simulink model "FullCarLateral"  (R2023b)
settings: Solver=FixedStepAuto  StartTime=0.0  StopTime=30  FixedStep=dt  MaxStep=0.001  RelTol=1e-3
model workspace (MAT data in the model file):
  AMU = Simulink.Signal
  AMU.DataType = 'double'
  AMU.Dimensions = 1
  AMU.DimensionsMode = 'auto'
  AMU.Complexity = 'real'
  AMU.SampleTime = -1
  AMU.SamplingMode = 'auto'
  EPSILON = Simulink.Signal
  EPSILON.DataType = 'double'
  EPSILON.Dimensions = 1
  EPSILON.DimensionsMode = 'auto'
  EPSILON.Complexity = 'real'
  EPSILON.SampleTime = -1
  EPSILON.SamplingMode = 'auto'
  FZO = Simulink.Signal
  FZO.DataType = 'double'
  FZO.Dimensions = 1
  FZO.DimensionsMode = 'auto'
  FZO.Complexity = 'real'
  FZO.SampleTime = -1
  FZO.SamplingMode = 'auto'
  LCX = Simulink.Signal
  LCX.DataType = 'double'
  LCX.Dimensions = 1
  LCX.DimensionsMode = 'auto'
  LCX.Complexity = 'real'
  LCX.SampleTime = -1
  LCX.SamplingMode = 'auto'
  LCY = Simulink.Signal
  LCY.DataType = 'double'
  LCY.Dimensions = 1
  LCY.DimensionsMode = 'auto'
  LCY.Complexity = 'real'
  LCY.SampleTime = -1
  LCY.SamplingMode = 'auto'
  LCZ = Simulink.Signal
  LCZ.DataType = 'double'
  LCZ.Dimensions = 1
  LCZ.DimensionsMode = 'auto'
  LCZ.Complexity = 'real'
  LCZ.SampleTime = -1
  LCZ.SamplingMode = 'auto'
  LEX = Simulink.Signal
  LEX.DataType = 'double'
  LEX.Dimensions = 1
  LEX.DimensionsMode = 'auto'
  LEX.Complexity = 'real'
  LEX.SampleTime = -1
  LEX.SamplingMode = 'auto'
  LEY = Simulink.Signal
  LEY.DataType = 'double'
  LEY.Dimensions = 1
  LEY.DimensionsMode = 'auto'
  LEY.Complexity = 'real'
  LEY.SampleTime = -1
  LEY.SamplingMode = 'auto'
  LFZO = Simulink.Signal
  LFZO.DataType = 'double'
  LFZO.Dimensions = 1
  LFZO.DimensionsMode = 'auto'
  LFZO.Complexity = 'real'
  LFZO.SampleTime = -1
  LFZO.SamplingMode = 'auto'
  LHX = Simulink.Signal
  LHX.DataType = 'double'
  LHX.Dimensions = 1
  LHX.DimensionsMode = 'auto'
  LHX.Complexity = 'real'
  LHX.SampleTime = -1
  LHX.SamplingMode = 'auto'
  LHY = Simulink.Signal
  LHY.DataType = 'double'
  LHY.Dimensions = 1
  LHY.DimensionsMode = 'auto'
  LHY.Complexity = 'real'
  LHY.SampleTime = -1
  LHY.SamplingMode = 'auto'
  LKXKAPPA = Simulink.Signal
  LKXKAPPA.DataType = 'double'
  LKXKAPPA.Dimensions = 1
  LKXKAPPA.DimensionsMode = 'auto'
  LKXKAPPA.Complexity = 'real'
  LKXKAPPA.SampleTime = -1
  LKXKAPPA.SamplingMode = 'auto'
  LKYALPHA = Simulink.Signal
  LKYALPHA.DataType = 'double'
  LKYALPHA.Dimensions = 1
  LKYALPHA.DimensionsMode = 'auto'
  LKYALPHA.Complexity = 'real'
  LKYALPHA.SampleTime = -1
  LKYALPHA.SamplingMode = 'auto'
  LKYGAMMA = Simulink.Signal
  LKYGAMMA.DataType = 'double'
  LKYGAMMA.Dimensions = 1
  LKYGAMMA.DimensionsMode = 'auto'
  LKYGAMMA.Complexity = 'real'
  LKYGAMMA.SampleTime = -1
  LKYGAMMA.SamplingMode = 'auto'
  LKZGAMMA = Simulink.Signal
  LKZGAMMA.DataType = 'double'
  LKZGAMMA.Dimensions = 1
  LKZGAMMA.DimensionsMode = 'auto'
  LKZGAMMA.Complexity = 'real'
  LKZGAMMA.SampleTime = -1
  LKZGAMMA.SamplingMode = 'auto'
  LMR = Simulink.Signal
  LMR.DataType = 'double'
  LMR.Dimensions = 1
  LMR.DimensionsMode = 'auto'
  LMR.Complexity = 'real'
  LMR.SampleTime = -1
  LMR.SamplingMode = 'auto'
  LMUV = Simulink.Signal
  LMUV.DataType = 'double'
  LMUV.Dimensions = 1
  LMUV.DimensionsMode = 'auto'
  LMUV.Complexity = 'real'
  LMUV.SampleTime = -1
  LMUV.SamplingMode = 'auto'
  LMUX = Simulink.Signal
  LMUX.DataType = 'double'
  LMUX.Dimensions = 1
  LMUX.DimensionsMode = 'auto'
  LMUX.Complexity = 'real'
  LMUX.SampleTime = -1
  LMUX.SamplingMode = 'auto'
  LMUXAST = Simulink.Signal
  LMUXAST.DataType = 'double'
  LMUXAST.Dimensions = 1
  LMUXAST.DimensionsMode = 'auto'
  LMUXAST.Complexity = 'real'
  LMUXAST.SampleTime = -1
  LMUXAST.SamplingMode = 'auto'
  LMUXPRIME = Simulink.Signal
  LMUXPRIME.DataType = 'double'
  LMUXPRIME.Dimensions = 1
  LMUXPRIME.DimensionsMode = 'auto'
  LMUXPRIME.Complexity = 'real'
  LMUXPRIME.SampleTime = -1
  LMUXPRIME.SamplingMode = 'auto'
  LMUY = Simulink.Signal
  LMUY.DataType = 'double'
  LMUY.Dimensions = 1
  LMUY.DimensionsMode = 'auto'
  LMUY.Complexity = 'real'
  LMUY.SampleTime = -1
  LMUY.SamplingMode = 'auto'
  LMUYAST = Simulink.Signal
  LMUYAST.DataType = 'double'
  LMUYAST.Dimensions = 1
  LMUYAST.DimensionsMode = 'auto'
  LMUYAST.Complexity = 'real'
  LMUYAST.SampleTime = -1
  LMUYAST.SamplingMode = 'auto'
  LMUYPRIME = Simulink.Signal
  LMUYPRIME.DataType = 'double'
  LMUYPRIME.Dimensions = 1
  LMUYPRIME.DimensionsMode = 'auto'
  LMUYPRIME.Complexity = 'real'
  LMUYPRIME.SampleTime = -1
  LMUYPRIME.SamplingMode = 'auto'
  LMX = Simulink.Signal
  LMX.DataType = 'double'
  LMX.Dimensions = 1
  LMX.DimensionsMode = 'auto'
  LMX.Complexity = 'real'
  LMX.SampleTime = -1
  LMX.SamplingMode = 'auto'
  LMY = Simulink.Signal
  LMY.DataType = 'double'
  LMY.Dimensions = 1
  LMY.DimensionsMode = 'auto'
  LMY.Complexity = 'real'
  LMY.SampleTime = -1
  LMY.SamplingMode = 'auto'
  LS = Simulink.Signal
  LS.DataType = 'double'
  LS.Dimensions = 1
  LS.DimensionsMode = 'auto'
  LS.Complexity = 'real'
  LS.SampleTime = -1
  LS.SamplingMode = 'auto'
  LT = Simulink.Signal
  LT.DataType = 'double'
  LT.Dimensions = 1
  LT.DimensionsMode = 'auto'
  LT.Complexity = 'real'
  LT.SampleTime = -1
  LT.SamplingMode = 'auto'
  LVX = Simulink.Signal
  LVX.DataType = 'double'
  LVX.Dimensions = 1
  LVX.DimensionsMode = 'auto'
  LVX.Complexity = 'real'
  LVX.SampleTime = -1
  LVX.SamplingMode = 'auto'
  LVY = Simulink.Signal
  LVY.DataType = 'double'
  LVY.Dimensions = 1
  LVY.DimensionsMode = 'auto'
  LVY.Complexity = 'real'
  LVY.SampleTime = -1
  LVY.SamplingMode = 'auto'
  LVYKAPPA = Simulink.Signal
  LVYKAPPA.DataType = 'double'
  LVYKAPPA.Dimensions = 1
  LVYKAPPA.DimensionsMode = 'auto'
  LVYKAPPA.Complexity = 'real'
  LVYKAPPA.SampleTime = -1
  LVYKAPPA.SamplingMode = 'auto'
  LXALPHA = Simulink.Signal
  LXALPHA.DataType = 'double'
  LXALPHA.Dimensions = 1
  LXALPHA.DimensionsMode = 'auto'
  LXALPHA.Complexity = 'real'
  LXALPHA.SampleTime = -1
  LXALPHA.SamplingMode = 'auto'
  LYKAPPA = Simulink.Signal
  LYKAPPA.DataType = 'double'
  LYKAPPA.Dimensions = 1
  LYKAPPA.DimensionsMode = 'auto'
  LYKAPPA.Complexity = 'real'
  LYKAPPA.SampleTime = -1
  LYKAPPA.SamplingMode = 'auto'
  PCX1 = Simulink.Signal
  PCX1.DataType = 'double'
  PCX1.Dimensions = 1
  PCX1.DimensionsMode = 'auto'
  PCX1.Complexity = 'real'
  PCX1.SampleTime = -1
  PCX1.SamplingMode = 'auto'
  PCY1 = Simulink.Signal
  PCY1.DataType = 'double'
  PCY1.Dimensions = 1
  PCY1.DimensionsMode = 'auto'
  PCY1.Complexity = 'real'
  PCY1.SampleTime = -1
  PCY1.SamplingMode = 'auto'
  PDX1 = Simulink.Signal
  PDX1.DataType = 'double'
  PDX1.Dimensions = 1
  PDX1.DimensionsMode = 'auto'
  PDX1.Complexity = 'real'
  PDX1.SampleTime = -1
  PDX1.SamplingMode = 'auto'
  PDX2 = Simulink.Signal
  PDX2.DataType = 'double'
  PDX2.Dimensions = 1
  PDX2.DimensionsMode = 'auto'
  PDX2.Complexity = 'real'
  PDX2.SampleTime = -1
  PDX2.SamplingMode = 'auto'
  PDX3 = Simulink.Signal
  PDX3.DataType = 'double'
  PDX3.Dimensions = 1
  PDX3.DimensionsMode = 'auto'
  PDX3.Complexity = 'real'
  PDX3.SampleTime = -1
  PDX3.SamplingMode = 'auto'
  PDY1 = Simulink.Signal
  PDY1.DataType = 'double'
  PDY1.Dimensions = 1
  PDY1.DimensionsMode = 'auto'
  PDY1.Complexity = 'real'
  PDY1.SampleTime = -1
  PDY1.SamplingMode = 'auto'
  PDY2 = Simulink.Signal
  PDY2.DataType = 'double'
  PDY2.Dimensions = 1
  PDY2.DimensionsMode = 'auto'
  PDY2.Complexity = 'real'
  PDY2.SampleTime = -1
  PDY2.SamplingMode = 'auto'
  PDY3 = Simulink.Signal
  PDY3.DataType = 'double'
  PDY3.Dimensions = 1
  PDY3.DimensionsMode = 'auto'
  PDY3.Complexity = 'real'
  PDY3.SampleTime = -1
  PDY3.SamplingMode = 'auto'
  PEX1 = Simulink.Signal
  PEX1.DataType = 'double'
  PEX1.Dimensions = 1
  PEX1.DimensionsMode = 'auto'
  PEX1.Complexity = 'real'
  PEX1.SampleTime = -1
  PEX1.SamplingMode = 'auto'
  PEX2 = Simulink.Signal
  PEX2.DataType = 'double'
  PEX2.Dimensions = 1
  PEX2.DimensionsMode = 'auto'
  PEX2.Complexity = 'real'
  PEX2.SampleTime = -1
  PEX2.SamplingMode = 'auto'
  PEX3 = Simulink.Signal
  PEX3.DataType = 'double'
  PEX3.Dimensions = 1
  PEX3.DimensionsMode = 'auto'
  PEX3.Complexity = 'real'
  PEX3.SampleTime = -1
  PEX3.SamplingMode = 'auto'
  PEX4 = Simulink.Signal
  PEX4.DataType = 'double'
  PEX4.Dimensions = 1
  PEX4.DimensionsMode = 'auto'
  PEX4.Complexity = 'real'
  PEX4.SampleTime = -1
  PEX4.SamplingMode = 'auto'
  PEY1 = Simulink.Signal
  PEY1.DataType = 'double'
  PEY1.Dimensions = 1
  PEY1.DimensionsMode = 'auto'
  PEY1.Complexity = 'real'
  PEY1.SampleTime = -1
  PEY1.SamplingMode = 'auto'
  PEY2 = Simulink.Signal
  PEY2.DataType = 'double'
  PEY2.Dimensions = 1
  PEY2.DimensionsMode = 'auto'
  PEY2.Complexity = 'real'
  PEY2.SampleTime = -1
  PEY2.SamplingMode = 'auto'
  PEY3 = Simulink.Signal
  PEY3.DataType = 'double'
  PEY3.Dimensions = 1
  PEY3.DimensionsMode = 'auto'
  PEY3.Complexity = 'real'
  PEY3.SampleTime = -1
  PEY3.SamplingMode = 'auto'
  PEY4 = Simulink.Signal
  PEY4.DataType = 'double'
  PEY4.Dimensions = 1
  PEY4.DimensionsMode = 'auto'
  PEY4.Complexity = 'real'
  PEY4.SampleTime = -1
  PEY4.SamplingMode = 'auto'
  PEY5 = Simulink.Signal
  PEY5.DataType = 'double'
  PEY5.Dimensions = 1
  PEY5.DimensionsMode = 'auto'
  PEY5.Complexity = 'real'
  PEY5.SampleTime = -1
  PEY5.SamplingMode = 'auto'
  PHX1 = Simulink.Signal
  PHX1.DataType = 'double'
  PHX1.Dimensions = 1
  PHX1.DimensionsMode = 'auto'
  PHX1.Complexity = 'real'
  PHX1.SampleTime = -1
  PHX1.SamplingMode = 'auto'
  PHX2 = Simulink.Signal
  PHX2.DataType = 'double'
  PHX2.Dimensions = 1
  PHX2.DimensionsMode = 'auto'
  PHX2.Complexity = 'real'
  PHX2.SampleTime = -1
  PHX2.SamplingMode = 'auto'
  PHY1 = Simulink.Signal
  PHY1.DataType = 'double'
  PHY1.Dimensions = 1
  PHY1.DimensionsMode = 'auto'
  PHY1.Complexity = 'real'
  PHY1.SampleTime = -1
  PHY1.SamplingMode = 'auto'
  PHY2 = Simulink.Signal
  PHY2.DataType = 'double'
  PHY2.Dimensions = 1
  PHY2.DimensionsMode = 'auto'
  PHY2.Complexity = 'real'
  PHY2.SampleTime = -1
  PHY2.SamplingMode = 'auto'
  PKX1 = Simulink.Signal
  PKX1.DataType = 'double'
  PKX1.Dimensions = 1
  PKX1.DimensionsMode = 'auto'
  PKX1.Complexity = 'real'
  PKX1.SampleTime = -1
  PKX1.SamplingMode = 'auto'
  PKX2 = Simulink.Signal
  PKX2.DataType = 'double'
  PKX2.Dimensions = 1
  PKX2.DimensionsMode = 'auto'
  PKX2.Complexity = 'real'
  PKX2.SampleTime = -1
  PKX2.SamplingMode = 'auto'
  PKX3 = Simulink.Signal
  PKX3.DataType = 'double'
  PKX3.Dimensions = 1
  PKX3.DimensionsMode = 'auto'
  PKX3.Complexity = 'real'
  PKX3.SampleTime = -1
  PKX3.SamplingMode = 'auto'
  PKY1 = Simulink.Signal
  PKY1.DataType = 'double'
  PKY1.Dimensions = 1
  PKY1.DimensionsMode = 'auto'
  PKY1.Complexity = 'real'
  PKY1.SampleTime = -1
  PKY1.SamplingMode = 'auto'
  PKY2 = Simulink.Signal
  PKY2.DataType = 'double'
  PKY2.Dimensions = 1
  PKY2.DimensionsMode = 'auto'
  PKY2.Complexity = 'real'
  PKY2.SampleTime = -1
  PKY2.SamplingMode = 'auto'
  PKY3 = Simulink.Signal
  PKY3.DataType = 'double'
  PKY3.Dimensions = 1
  PKY3.DimensionsMode = 'auto'
  PKY3.Complexity = 'real'
  PKY3.SampleTime = -1
  PKY3.SamplingMode = 'auto'
  PKY4 = Simulink.Signal
  PKY4.DataType = 'double'
  PKY4.Dimensions = 1
  PKY4.DimensionsMode = 'auto'
  PKY4.Complexity = 'real'
  PKY4.SampleTime = -1
  PKY4.SamplingMode = 'auto'
  PKY5 = Simulink.Signal
  PKY5.DataType = 'double'
  PKY5.Dimensions = 1
  PKY5.DimensionsMode = 'auto'
  PKY5.Complexity = 'real'
  PKY5.SampleTime = -1
  PKY5.SamplingMode = 'auto'
  PKY6 = Simulink.Signal
  PKY6.DataType = 'double'
  PKY6.Dimensions = 1
  PKY6.DimensionsMode = 'auto'
  PKY6.Complexity = 'real'
  PKY6.SampleTime = -1
  PKY6.SamplingMode = 'auto'
  PKY7 = Simulink.Signal
  PKY7.DataType = 'double'
  PKY7.Dimensions = 1
  PKY7.DimensionsMode = 'auto'
  PKY7.Complexity = 'real'
  PKY7.SampleTime = -1
  PKY7.SamplingMode = 'auto'
  PVX1 = Simulink.Signal
  PVX1.DataType = 'double'
  PVX1.Dimensions = 1
  PVX1.DimensionsMode = 'auto'
  PVX1.Complexity = 'real'
  PVX1.SampleTime = -1
  PVX1.SamplingMode = 'auto'
  PVX2 = Simulink.Signal
  PVX2.DataType = 'double'
  PVX2.Dimensions = 1
  PVX2.DimensionsMode = 'auto'
  PVX2.Complexity = 'real'
  PVX2.SampleTime = -1
  PVX2.SamplingMode = 'auto'
  PVY1 = Simulink.Signal
  PVY1.DataType = 'double'
  PVY1.Dimensions = 1
  PVY1.DimensionsMode = 'auto'
  PVY1.Complexity = 'real'
  PVY1.SampleTime = -1
  PVY1.SamplingMode = 'auto'
  PVY2 = Simulink.Signal
  PVY2.DataType = 'double'
  PVY2.Dimensions = 1
  PVY2.DimensionsMode = 'auto'
  PVY2.Complexity = 'real'
  PVY2.SampleTime = -1
  PVY2.SamplingMode = 'auto'
  PVY3 = Simulink.Signal
  PVY3.DataType = 'double'
  PVY3.Dimensions = 1
  PVY3.DimensionsMode = 'auto'
  PVY3.Complexity = 'real'
  PVY3.SampleTime = -1
  PVY3.SamplingMode = 'auto'
  PVY4 = Simulink.Signal
  PVY4.DataType = 'double'
  PVY4.Dimensions = 1
  PVY4.DimensionsMode = 'auto'
  PVY4.Complexity = 'real'
  PVY4.SampleTime = -1
  PVY4.SamplingMode = 'auto'
  QBZ1 = Simulink.Signal
  QBZ1.DataType = 'double'
  QBZ1.Dimensions = 1
  QBZ1.DimensionsMode = 'auto'
  QBZ1.Complexity = 'real'
  QBZ1.SampleTime = -1
  QBZ1.SamplingMode = 'auto'
  QBZ10 = Simulink.Signal
  QBZ10.DataType = 'double'
  QBZ10.Dimensions = 1
  QBZ10.DimensionsMode = 'auto'
  QBZ10.Complexity = 'real'
  QBZ10.SampleTime = -1
  QBZ10.SamplingMode = 'auto'
  QBZ2 = Simulink.Signal
  QBZ2.DataType = 'double'
  QBZ2.Dimensions = 1
  QBZ2.DimensionsMode = 'auto'
  QBZ2.Complexity = 'real'
  QBZ2.SampleTime = -1
  QBZ2.SamplingMode = 'auto'
  QBZ3 = Simulink.Signal
  QBZ3.DataType = 'double'
  QBZ3.Dimensions = 1
  QBZ3.DimensionsMode = 'auto'
  QBZ3.Complexity = 'real'
  QBZ3.SampleTime = -1
  QBZ3.SamplingMode = 'auto'
  QBZ5 = Simulink.Signal
  QBZ5.DataType = 'double'
  QBZ5.Dimensions = 1
  QBZ5.DimensionsMode = 'auto'
  QBZ5.Complexity = 'real'
  QBZ5.SampleTime = -1
  QBZ5.SamplingMode = 'auto'
  QBZ6 = Simulink.Signal
  QBZ6.DataType = 'double'
  QBZ6.Dimensions = 1
  QBZ6.DimensionsMode = 'auto'
  QBZ6.Complexity = 'real'
  QBZ6.SampleTime = -1
  QBZ6.SamplingMode = 'auto'
  QBZ9 = Simulink.Signal
  QBZ9.DataType = 'double'
  QBZ9.Dimensions = 1
  QBZ9.DimensionsMode = 'auto'
  QBZ9.Complexity = 'real'
  QBZ9.SampleTime = -1
  QBZ9.SamplingMode = 'auto'
  QCZ1 = Simulink.Signal
  QCZ1.DataType = 'double'
  QCZ1.Dimensions = 1
  QCZ1.DimensionsMode = 'auto'
  QCZ1.Complexity = 'real'
  QCZ1.SampleTime = -1
  QCZ1.SamplingMode = 'auto'
  QDZ1 = Simulink.Signal
  QDZ1.DataType = 'double'
  QDZ1.Dimensions = 1
  QDZ1.DimensionsMode = 'auto'
  QDZ1.Complexity = 'real'
  QDZ1.SampleTime = -1
  QDZ1.SamplingMode = 'auto'
  QDZ10 = Simulink.Signal
  QDZ10.DataType = 'double'
  QDZ10.Dimensions = 1
  QDZ10.DimensionsMode = 'auto'
  QDZ10.Complexity = 'real'
  QDZ10.SampleTime = -1
  QDZ10.SamplingMode = 'auto'
  QDZ11 = Simulink.Signal
  QDZ11.DataType = 'double'
  QDZ11.Dimensions = 1
  QDZ11.DimensionsMode = 'auto'
  QDZ11.Complexity = 'real'
  QDZ11.SampleTime = -1
  QDZ11.SamplingMode = 'auto'
  QDZ2 = Simulink.Signal
  QDZ2.DataType = 'double'
  QDZ2.Dimensions = 1
  QDZ2.DimensionsMode = 'auto'
  QDZ2.Complexity = 'real'
  QDZ2.SampleTime = -1
  QDZ2.SamplingMode = 'auto'
  QDZ3 = Simulink.Signal
  QDZ3.DataType = 'double'
  QDZ3.Dimensions = 1
  QDZ3.DimensionsMode = 'auto'
  QDZ3.Complexity = 'real'
  QDZ3.SampleTime = -1
  QDZ3.SamplingMode = 'auto'
  QDZ4 = Simulink.Signal
  QDZ4.DataType = 'double'
  QDZ4.Dimensions = 1
  QDZ4.DimensionsMode = 'auto'
  QDZ4.Complexity = 'real'
  QDZ4.SampleTime = -1
  QDZ4.SamplingMode = 'auto'
  QDZ6 = Simulink.Signal
  QDZ6.DataType = 'double'
  QDZ6.Dimensions = 1
  QDZ6.DimensionsMode = 'auto'
  QDZ6.Complexity = 'real'
  QDZ6.SampleTime = -1
  QDZ6.SamplingMode = 'auto'
  QDZ7 = Simulink.Signal
  QDZ7.DataType = 'double'
  QDZ7.Dimensions = 1
  QDZ7.DimensionsMode = 'auto'
  QDZ7.Complexity = 'real'
  QDZ7.SampleTime = -1
  QDZ7.SamplingMode = 'auto'
  QDZ8 = Simulink.Signal
  QDZ8.DataType = 'double'
  QDZ8.Dimensions = 1
  QDZ8.DimensionsMode = 'auto'
  QDZ8.Complexity = 'real'
  QDZ8.SampleTime = -1
  QDZ8.SamplingMode = 'auto'
  QDZ9 = Simulink.Signal
  QDZ9.DataType = 'double'
  QDZ9.Dimensions = 1
  QDZ9.DimensionsMode = 'auto'
  QDZ9.Complexity = 'real'
  QDZ9.SampleTime = -1
  QDZ9.SamplingMode = 'auto'
  QEZ1 = Simulink.Signal
  QEZ1.DataType = 'double'
  QEZ1.Dimensions = 1
  QEZ1.DimensionsMode = 'auto'
  QEZ1.Complexity = 'real'
  QEZ1.SampleTime = -1
  QEZ1.SamplingMode = 'auto'
  QEZ2 = Simulink.Signal
  QEZ2.DataType = 'double'
  QEZ2.Dimensions = 1
  QEZ2.DimensionsMode = 'auto'
  QEZ2.Complexity = 'real'
  QEZ2.SampleTime = -1
  QEZ2.SamplingMode = 'auto'
  QEZ3 = Simulink.Signal
  QEZ3.DataType = 'double'
  QEZ3.Dimensions = 1
  QEZ3.DimensionsMode = 'auto'
  QEZ3.Complexity = 'real'
  QEZ3.SampleTime = -1
  QEZ3.SamplingMode = 'auto'
  QEZ4 = Simulink.Signal
  QEZ4.DataType = 'double'
  QEZ4.Dimensions = 1
  QEZ4.DimensionsMode = 'auto'
  QEZ4.Complexity = 'real'
  QEZ4.SampleTime = -1
  QEZ4.SamplingMode = 'auto'
  QEZ5 = Simulink.Signal
  QEZ5.DataType = 'double'
  QEZ5.Dimensions = 1
  QEZ5.DimensionsMode = 'auto'
  QEZ5.Complexity = 'real'
  QEZ5.SampleTime = -1
  QEZ5.SamplingMode = 'auto'
  QHZ1 = Simulink.Signal
  QHZ1.DataType = 'double'
  QHZ1.Dimensions = 1
  QHZ1.DimensionsMode = 'auto'
  QHZ1.Complexity = 'real'
  QHZ1.SampleTime = -1
  QHZ1.SamplingMode = 'auto'
  QHZ2 = Simulink.Signal
  QHZ2.DataType = 'double'
  QHZ2.Dimensions = 1
  QHZ2.DimensionsMode = 'auto'
  QHZ2.Complexity = 'real'
  QHZ2.SampleTime = -1
  QHZ2.SamplingMode = 'auto'
  QHZ3 = Simulink.Signal
  QHZ3.DataType = 'double'
  QHZ3.Dimensions = 1
  QHZ3.DimensionsMode = 'auto'
  QHZ3.Complexity = 'real'
  QHZ3.SampleTime = -1
  QHZ3.SamplingMode = 'auto'
  QHZ4 = Simulink.Signal
  QHZ4.DataType = 'double'
  QHZ4.Dimensions = 1
  QHZ4.DimensionsMode = 'auto'
  QHZ4.Complexity = 'real'
  QHZ4.SampleTime = -1
  QHZ4.SamplingMode = 'auto'
  QSX1 = Simulink.Signal
  QSX1.DataType = 'double'
  QSX1.Dimensions = 1
  QSX1.DimensionsMode = 'auto'
  QSX1.Complexity = 'real'
  QSX1.SampleTime = -1
  QSX1.SamplingMode = 'auto'
  QSX2 = Simulink.Signal
  QSX2.DataType = 'double'
  QSX2.Dimensions = 1
  QSX2.DimensionsMode = 'auto'
  QSX2.Complexity = 'real'
  QSX2.SampleTime = -1
  QSX2.SamplingMode = 'auto'
  QSX3 = Simulink.Signal
  QSX3.DataType = 'double'
  QSX3.Dimensions = 1
  QSX3.DimensionsMode = 'auto'
  QSX3.Complexity = 'real'
  QSX3.SampleTime = -1
  QSX3.SamplingMode = 'auto'
  QX1 = Simulink.Signal
  QX1.DataType = 'double'
  QX1.Dimensions = 1
  QX1.DimensionsMode = 'auto'
  QX1.Complexity = 'real'
  QX1.SampleTime = -1
  QX1.SamplingMode = 'auto'
  QX2 = Simulink.Signal
  QX2.DataType = 'double'
  QX2.Dimensions = 1
  QX2.DimensionsMode = 'auto'
  QX2.Complexity = 'real'
  QX2.SampleTime = -1
  QX2.SamplingMode = 'auto'
  QX3 = Simulink.Signal
  QX3.DataType = 'double'
  QX3.Dimensions = 1
  QX3.DimensionsMode = 'auto'
  QX3.Complexity = 'real'
  QX3.SampleTime = -1
  QX3.SamplingMode = 'auto'
  QX4 = Simulink.Signal
  QX4.DataType = 'double'
  QX4.Dimensions = 1
  QX4.DimensionsMode = 'auto'
  QX4.Complexity = 'real'
  QX4.SampleTime = -1
  QX4.SamplingMode = 'auto'
  QX5 = Simulink.Signal
  QX5.DataType = 'double'
  QX5.Dimensions = 1
  QX5.DimensionsMode = 'auto'
  QX5.Complexity = 'real'
  QX5.SampleTime = -1
  QX5.SamplingMode = 'auto'
  QX6 = Simulink.Signal
  QX6.DataType = 'double'
  QX6.Dimensions = 1
  QX6.DimensionsMode = 'auto'
  QX6.Complexity = 'real'
  QX6.SampleTime = -1
  QX6.SamplingMode = 'auto'
  RBX1 = Simulink.Signal
  RBX1.DataType = 'double'
  RBX1.Dimensions = 1
  RBX1.DimensionsMode = 'auto'
  RBX1.Complexity = 'real'
  RBX1.SampleTime = -1
  RBX1.SamplingMode = 'auto'
  RBX2 = Simulink.Signal
  RBX2.DataType = 'double'
  RBX2.Dimensions = 1
  RBX2.DimensionsMode = 'auto'
  RBX2.Complexity = 'real'
  RBX2.SampleTime = -1
  RBX2.SamplingMode = 'auto'
  RBX3 = Simulink.Signal
  RBX3.DataType = 'double'
  RBX3.Dimensions = 1
  RBX3.DimensionsMode = 'auto'
  RBX3.Complexity = 'real'
  RBX3.SampleTime = -1
  RBX3.SamplingMode = 'auto'
  RBY1 = Simulink.Signal
  RBY1.DataType = 'double'
  RBY1.Dimensions = 1
  RBY1.DimensionsMode = 'auto'
  RBY1.Complexity = 'real'
  RBY1.SampleTime = -1
  RBY1.SamplingMode = 'auto'
  RBY2 = Simulink.Signal
  RBY2.DataType = 'double'
  RBY2.Dimensions = 1
  RBY2.DimensionsMode = 'auto'
  RBY2.Complexity = 'real'
  RBY2.SampleTime = -1
  RBY2.SamplingMode = 'auto'
  RBY3 = Simulink.Signal
  RBY3.DataType = 'double'
  RBY3.Dimensions = 1
  RBY3.DimensionsMode = 'auto'
  RBY3.Complexity = 'real'
  RBY3.SampleTime = -1
  RBY3.SamplingMode = 'auto'
  RBY4 = Simulink.Signal
  RBY4.DataType = 'double'
  RBY4.Dimensions = 1
  RBY4.DimensionsMode = 'auto'
  RBY4.Complexity = 'real'
  RBY4.SampleTime = -1
  RBY4.SamplingMode = 'auto'
  RCX1 = Simulink.Signal
  RCX1.DataType = 'double'
  RCX1.Dimensions = 1
  RCX1.DimensionsMode = 'auto'
  RCX1.Complexity = 'real'
  RCX1.SampleTime = -1
  RCX1.SamplingMode = 'auto'
  RCY1 = Simulink.Signal
  RCY1.DataType = 'double'
  RCY1.Dimensions = 1
  RCY1.DimensionsMode = 'auto'
  RCY1.Complexity = 'real'
  RCY1.SampleTime = -1
  RCY1.SamplingMode = 'auto'
  REX1 = Simulink.Signal
  REX1.DataType = 'double'
  REX1.Dimensions = 1
  REX1.DimensionsMode = 'auto'
  REX1.Complexity = 'real'
  REX1.SampleTime = -1
  REX1.SamplingMode = 'auto'
  REX2 = Simulink.Signal
  REX2.DataType = 'double'
  REX2.Dimensions = 1
  REX2.DimensionsMode = 'auto'
  REX2.Complexity = 'real'
  REX2.SampleTime = -1
  REX2.SamplingMode = 'auto'
  REY1 = Simulink.Signal
  REY1.DataType = 'double'
  REY1.Dimensions = 1
  REY1.DimensionsMode = 'auto'
  REY1.Complexity = 'real'
  REY1.SampleTime = -1
  REY1.SamplingMode = 'auto'
  REY2 = Simulink.Signal
  REY2.DataType = 'double'
  REY2.Dimensions = 1
  REY2.DimensionsMode = 'auto'
  REY2.Complexity = 'real'
  REY2.SampleTime = -1
  REY2.SamplingMode = 'auto'
  RHX1 = Simulink.Signal
  RHX1.DataType = 'double'
  RHX1.Dimensions = 1
  RHX1.DimensionsMode = 'auto'
  RHX1.Complexity = 'real'
  RHX1.SampleTime = -1
  RHX1.SamplingMode = 'auto'
  RHY1 = Simulink.Signal
  RHY1.DataType = 'double'
  RHY1.Dimensions = 1
  RHY1.DimensionsMode = 'auto'
  RHY1.Complexity = 'real'
  RHY1.SampleTime = -1
  RHY1.SamplingMode = 'auto'
  RHY2 = Simulink.Signal
  RHY2.DataType = 'double'
  RHY2.Dimensions = 1
  RHY2.DimensionsMode = 'auto'
  RHY2.Complexity = 'real'
  RHY2.SampleTime = -1
  RHY2.SamplingMode = 'auto'
  RO = Simulink.Signal
  RO.DataType = 'double'
  RO.Dimensions = 1
  RO.DimensionsMode = 'auto'
  RO.Complexity = 'real'
  RO.SampleTime = -1
  RO.SamplingMode = 'auto'
  RVY1 = Simulink.Signal
  RVY1.DataType = 'double'
  RVY1.Dimensions = 1
  RVY1.DimensionsMode = 'auto'
  RVY1.Complexity = 'real'
  RVY1.SampleTime = -1
  RVY1.SamplingMode = 'auto'
  RVY2 = Simulink.Signal
  RVY2.DataType = 'double'
  RVY2.Dimensions = 1
  RVY2.DimensionsMode = 'auto'
  RVY2.Complexity = 'real'
  RVY2.SampleTime = -1
  RVY2.SamplingMode = 'auto'
  RVY3 = Simulink.Signal
  RVY3.DataType = 'double'
  RVY3.Dimensions = 1
  RVY3.DimensionsMode = 'auto'
  RVY3.Complexity = 'real'
  RVY3.SampleTime = -1
  RVY3.SamplingMode = 'auto'
  RVY4 = Simulink.Signal
  RVY4.DataType = 'double'
  RVY4.Dimensions = 1
  RVY4.DimensionsMode = 'auto'
  RVY4.Complexity = 'real'
  RVY4.SampleTime = -1
  RVY4.SamplingMode = 'auto'
  RVY5 = Simulink.Signal
  RVY5.DataType = 'double'
  RVY5.Dimensions = 1
  RVY5.DimensionsMode = 'auto'
  RVY5.Complexity = 'real'
  RVY5.SampleTime = -1
  RVY5.SamplingMode = 'auto'
  RVY6 = Simulink.Signal
  RVY6.DataType = 'double'
  RVY6.Dimensions = 1
  RVY6.DimensionsMode = 'auto'
  RVY6.Complexity = 'real'
  RVY6.SampleTime = -1
  RVY6.SamplingMode = 'auto'
  SSZ1 = Simulink.Signal
  SSZ1.DataType = 'double'
  SSZ1.Dimensions = 1
  SSZ1.DimensionsMode = 'auto'
  SSZ1.Complexity = 'real'
  SSZ1.SampleTime = -1
  SSZ1.SamplingMode = 'auto'
  SSZ2 = Simulink.Signal
  SSZ2.DataType = 'double'
  SSZ2.Dimensions = 1
  SSZ2.DimensionsMode = 'auto'
  SSZ2.Complexity = 'real'
  SSZ2.SampleTime = -1
  SSZ2.SamplingMode = 'auto'
  SSZ3 = Simulink.Signal
  SSZ3.DataType = 'double'
  SSZ3.Dimensions = 1
  SSZ3.DimensionsMode = 'auto'
  SSZ3.Complexity = 'real'
  SSZ3.SampleTime = -1
  SSZ3.SamplingMode = 'auto'
  SSZ4 = Simulink.Signal
  SSZ4.DataType = 'double'
  SSZ4.Dimensions = 1
  SSZ4.DimensionsMode = 'auto'
  SSZ4.Complexity = 'real'
  SSZ4.SampleTime = -1
  SSZ4.SamplingMode = 'auto'
  VCX = Simulink.Signal
  VCX.DataType = 'double'
  VCX.Dimensions = 1
  VCX.DimensionsMode = 'auto'
  VCX.Complexity = 'real'
  VCX.SampleTime = -1
  VCX.SamplingMode = 'auto'
  ZETA0 = Simulink.Signal
  ZETA0.DataType = 'double'
  ZETA0.Dimensions = 1
  ZETA0.DimensionsMode = 'auto'
  ZETA0.Complexity = 'real'
  ZETA0.SampleTime = -1
  ZETA0.SamplingMode = 'auto'
  ZETA1 = Simulink.Signal
  ZETA1.DataType = 'double'
  ZETA1.Dimensions = 1
  ZETA1.DimensionsMode = 'auto'
  ZETA1.Complexity = 'real'
  ZETA1.SampleTime = -1
  ZETA1.SamplingMode = 'auto'
  ZETA2 = Simulink.Signal
  ZETA2.DataType = 'double'
  ZETA2.Dimensions = 1
  ZETA2.DimensionsMode = 'auto'
  ZETA2.Complexity = 'real'
  ZETA2.SampleTime = -1
  ZETA2.SamplingMode = 'auto'
  ZETA3 = Simulink.Signal
  ZETA3.DataType = 'double'
  ZETA3.Dimensions = 1
  ZETA3.DimensionsMode = 'auto'
  ZETA3.Complexity = 'real'
  ZETA3.SampleTime = -1
  ZETA3.SamplingMode = 'auto'
  ZETA4 = Simulink.Signal
  ZETA4.DataType = 'double'
  ZETA4.Dimensions = 1
  ZETA4.DimensionsMode = 'auto'
  ZETA4.Complexity = 'real'
  ZETA4.SampleTime = -1
  ZETA4.SamplingMode = 'auto'
  ZETA5 = Simulink.Signal
  ZETA5.DataType = 'double'
  ZETA5.Dimensions = 1
  ZETA5.DimensionsMode = 'auto'
  ZETA5.Complexity = 'real'
  ZETA5.SampleTime = -1
  ZETA5.SamplingMode = 'auto'
  ZETA6 = Simulink.Signal
  ZETA6.DataType = 'double'
  ZETA6.Dimensions = 1
  ZETA6.DimensionsMode = 'auto'
  ZETA6.Complexity = 'real'
  ZETA6.SampleTime = -1
  ZETA6.SamplingMode = 'auto'
  ZETA7 = Simulink.Signal
  ZETA7.DataType = 'double'
  ZETA7.Dimensions = 1
  ZETA7.DimensionsMode = 'auto'
  ZETA7.Complexity = 'real'
  ZETA7.SampleTime = -1
  ZETA7.SamplingMode = 'auto'
  ZETA8 = Simulink.Signal
  ZETA8.DataType = 'double'
  ZETA8.Dimensions = 1
  ZETA8.DimensionsMode = 'auto'
  ZETA8.Complexity = 'real'
  ZETA8.SampleTime = -1
  ZETA8.SamplingMode = 'auto'
values from neighbouring files (symbols this model uses):
  A = load('PSS LATERAL FORCE COEFFS.mat').A    [FullCarLateralParams.m]
  B = load('PSS ALIGNING TORQUE COEFFS.mat').B    [FullCarLateralParams.m]
  b = 0.085    [FullCarLateralParams.m]
  C = load('COMBINED OVERTURNING MOMENT COEFFS.mat').C    [FullCarLateralParams.m]
  c_roll = 0.1    [FullCarLateralParams.m]
  cD = 1.23    [FullCarLateralParams.m]
  cL = 3.71    [FullCarLateralParams.m]
  D = load('PLS LONGITUDINAL FORCE COEFFS.mat').D    [FullCarLateralParams.m]
  dt = 0.001    [FullCarLateralParams.m]
  E = load('COMBINED LONGITUDINAL FORCE COEFFS.mat').E    [FullCarLateralParams.m]
  e_FL = atan(tf/lf)    [FullCarLateralParams.m]
  e_FR = atan(lf/tf)    [FullCarLateralParams.m]
  e_RL = atan(lr/tr)    [FullCarLateralParams.m]
  e_RR = atan(tr/lr)    [FullCarLateralParams.m]
  F = load('COMBINED LATERAL FORCE COEFFS.mat').F    [FullCarLateralParams.m]
  frontalA = 1    [FullCarLateralParams.m]
  g = 9.81    [FullCarLateralParams.m]
  G = load('COMBINED ALIGNING TORQUE COEFFS.mat').G    [FullCarLateralParams.m]
  gearboxEff = 0.95    [FullCarLateralParams.m]
  GR = 11.86    [FullCarLateralParams.m]
  hCG = 0.2    [FullCarLateralParams.m]
  Ix_wheel = (0.07829 + Ix_motor*GR*GR) * Ix_wheel_factor    (= 0.1168307304)    [FullCarLateralParams.m]
  Iz_vehicle = 125    [FullCarLateralParams.m]
  lf = wb - lr    (= 0.755)    [FullCarLateralParams.m]
  lowpassT = 0.05    [FullCarLateralParams.m]
  lr = 0.78    [FullCarLateralParams.m]
  m = 250    [FullCarLateralParams.m]
  motorOmegaLimit = 2094    [FullCarLateralParams.m]
  R_FL = sqrt(tf^2 + lf^2)    [FullCarLateralParams.m]
  R_FR = R_FL    [FullCarLateralParams.m]
  R_RL = sqrt(tr^2 + lr^2)    [FullCarLateralParams.m]
  R_RR = R_RL    [FullCarLateralParams.m]
  R_wheel = 0.2    [FullCarLateralParams.m]
  rho = 1.293    [FullCarLateralParams.m]
  tireFactor_X_Accel = 0.6    [FullCarLateralParams.m]
  tireFactor_X_Brake = 0.6    [FullCarLateralParams.m]
  tireFactor_Y = 1    [FullCarLateralParams.m]
  TLLTD = 0.5    [FullCarLateralParams.m]
  tr = trackWidth / 2    (= 0.6)    [FullCarLateralParams.m]
  trackWidth = 1.2    [FullCarLateralParams.m]
  wb = 1.535    [FullCarLateralParams.m]
  wheelSideBrakeFactor = 1    [FullCarLateralParams.m]
undefined symbols (not defined in the file or in its folder): trackReference
libraries: simulink_extras x11, eeGeneralControl x3, slpidlib x2, simulink x2
(part 1 of 6)
settings Model: PauseTimes=0  PacingRate=0.010000  Creator=lukec  LastModifiedBy=ben
settings OptimizationCC: DefaultParameterBehavior=Inlined  EnhancedBackFolding=on  PassReuseOutputArgsAs=Individual arguments  ZeroExternalMemoryAtStartup=off  ZeroInternalMemoryAtStartup=off  OptimizeBlockOrder=speed  DifferentSizesBufferReuse=on  OptimizationCustomize=off  EfficientTunableParamExpr=on
settings DebuggingCC: ParameterTunabilityLossMsg=error
settings SFSimCC: MATLABDynamicMemAlloc=off
settings RTWCC: Description=Embedded Coder  SystemTargetFile=ert.tlc  GenCodeOnly=on  PackageGeneratedCodeAndArtifacts=on  TemplateMakefile=ert_default_tmf  GenerateReport=on  Toolchain=CMake  TargetLang=C++
settings CodeAppCC: ForceParamTrailComments=on  IgnoreCustomStorageClasses=off  OperatorAnnotations=on  SimulinkDataObjDesc=on  SFDataObjDesc=on  InsertBlockDesc=on
settings ERTTargetCC: TargetLangStandard=C++11 (ISO)  GenerateSampleERTMain=on  CodeInterfacePackaging=C++ class  InlinedParameterPlacement=NonHierarchical  RootIOFormat=Structure reference  ERTCustomFileTemplate=example_file_process.tlc

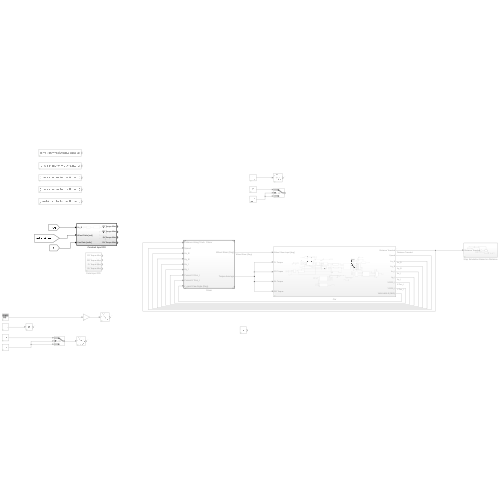
[thumbnail: Simulink's stored preview of the top-level diagram]
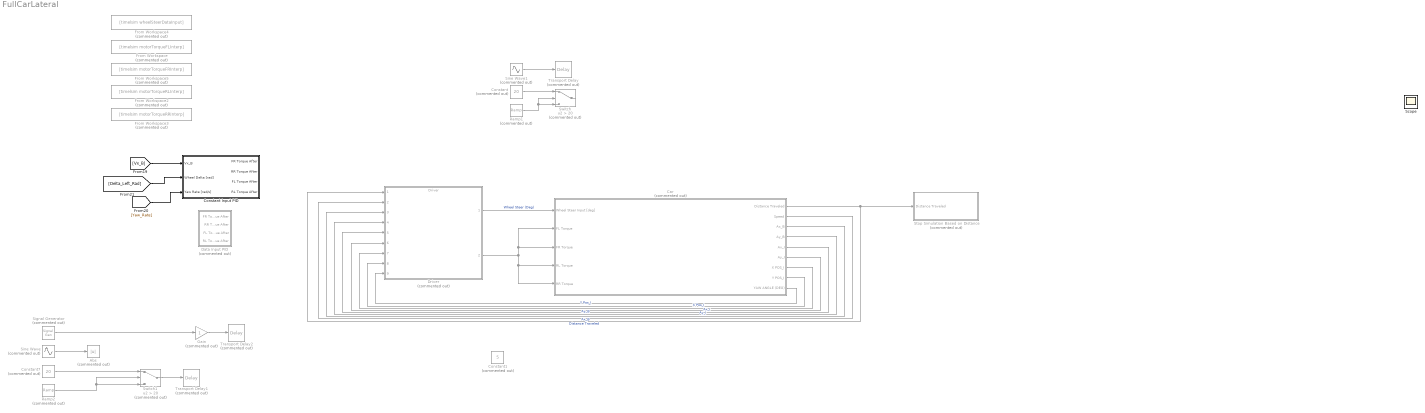
== system FullCarLateral ==
  Abs : Abs  Commented=on  SaturateOnIntegerOverflow=off
  Car : Subsystem  Commented=on
  Constant : Constant  Commented=on  Value=20
  Constant Input PID : Subsystem  TreatAsAtomicUnit=on
  Constant1 : Constant  Commented=on  Value=5
  Constant7 : Constant  Commented=on  Value=20
  Data Input PID : Subsystem  Commented=on
  Driver : ModelReference  Commented=on  ModelNameDialog=Driver  SimulationMode=Normal  ModelReferenceVersion=1.11
  From Workspace : FromWorkspace  Commented=on  VariableName=[timelsim motorTorqueFLInterp]
  From Workspace2 : FromWorkspace  Commented=on  VariableName=[timelsim motorTorqueRLInterp]
  From Workspace3 : FromWorkspace  Commented=on  VariableName=[timelsim motorTorqueRRInterp]
  From Workspace4 : FromWorkspace  Commented=on  VariableName=[timelsim wheelSteerDataInput]
  From Workspace5 : FromWorkspace  Commented=on  VariableName=[timelsim motorTorqueFRInterp]
  Gain : Gain  Commented=on
  Ramp1 : simulink/Sources/Ramp  Commented=on  slope=20  start=0  InitialOutput=0
  Ramp2 : simulink/Sources/Ramp  Commented=on  slope=0  start=0  InitialOutput=0
  Signal Generator : SignalGenerator  Commented=on  Amplitude=5  Frequency=.125  Units=rad/sec
  Sine Wave : Sin  Commented=on  Amplitude=5  Frequency=.25  SampleTime=0
  Sine Wave1 : Sin  Commented=on  Amplitude=10  SampleTime=0
  Stop Simulation Based on Distance : Subsystem  Commented=on
  Switch : Switch  Commented=on  Criteria=u2 > Threshold  Threshold=20  SaturateOnIntegerOverflow=off  InputSameDT=off
  Switch1 : Switch  Commented=on  Criteria=u2 > Threshold  Threshold=20  SaturateOnIntegerOverflow=off  InputSameDT=off
  Transport Delay : TransportDelay  Commented=on  DelayTime=2  BufferSize=10240
  Transport Delay1 : TransportDelay  Commented=on  DelayTime=5  BufferSize=10240
  Transport Delay2 : TransportDelay  Commented=on  DelayTime=5  BufferSize=10240
  Scope : Scope
  wires:
  [Yaw_Rate] -> Constant Input PID/3(Yaw Rate [rad/s])
  [Vx_B] -> Constant Input PID/1(Vx_B)
  Sine Wave/1 -> Abs/1
  Sine Wave1/1 -> Transport Delay/1
  Constant/1 -> Switch/1
  Ramp1/1 -> Switch/3, Switch/2
  [Delta_Left_Rad] -> Constant Input PID/2(Wheel Delta [rad])
  Ramp2/1 -> Switch1/2, Switch1/3
  Signal Generator/1 -> Gain/1
  Constant7/1 -> Switch1/1
  Car/1(Distance Traveled) -> Driver/1, Stop Simulation Based on Distance/1(Distance Traveled)  "Distance Traveled"
  Car/2(Speed) -> Driver/2
  Car/4(Ay_B) -> Driver/4  "Ay_B"
  Car/3(Ax_B) -> Driver/3  "Ax_B"
  Switch1/1 -> Transport Delay1/1
  Car/6(Ay_I) -> Driver/6  "Ay_I"
  Car/5(Ax_I) -> Driver/5  "Ax_I"
  Car/8(Y POS_I) -> Driver/8  "Y Pos_I"
  Car/7(X POS_I) -> Driver/7  "X Pos_I"
  Car/9(YAW ANGLE (DEG)) -> Driver/9
  Gain/1 -> Transport Delay2/1
  Driver/1 -> Car/1(Wheel Steer Input [deg])  "Wheel Steer (Deg)"
  Driver/2 -> Car/5(RR Torque), Car/4(RL Torque), Car/3(FR Torque), Car/2(FL Torque)

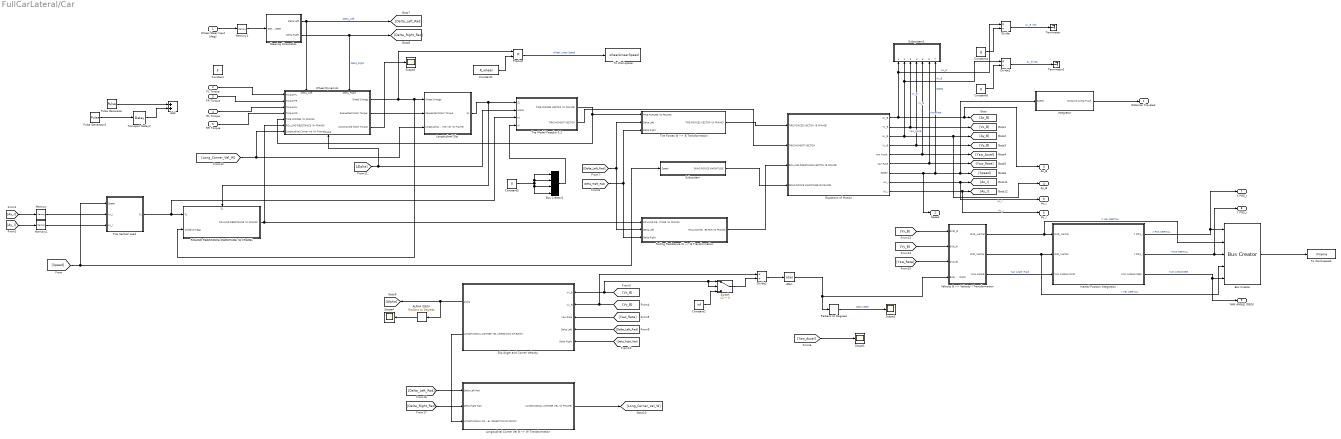
== system FullCarLateral/Car ==
  Wheel Steer Input [deg] : Inport
  FL Torque : Inport  Port=2
  FR Torque : Inport  Port=3
  RL Torque : Inport  Port=4
  RR Torque : Inport  Port=5
  ALPHA (DEG) : simulink_extras/Transformations/Radians to Degrees
  Add : Sum
  Atan : Trigonometry  Operator=atan
  Bus Creator : BusCreator  Inputs=5
  Bus Creator1 : BusCreator  Inputs=4
  Constant : Constant  Value=5
  Constant1 : Constant  Value=R_wheel
  Constant2 : Constant  Value=inf
  Constant4 : Constant  Value=g
  Constant5 : Constant  Value=0
  Constant6 : Constant  Value=g
  Divide : Product  Inputs=*/
  Divide1 : Product  Inputs=*/
  Divide2 : Product  Inputs=*/
  Equations of Motion : Subsystem
  Inertial Position Integration : Subsystem
  Integrator : Subsystem
  Longitudinal Corner Vel B --> W Transformation : Subsystem
  Longitudinal Slip : Subsystem
  Memory : Memory
  Memory1 : Memory
  Memory2 : Memory
  Product : Product
  Pulse Generator : DiscretePulseGenerator  PulseType=Time based  Amplitude=20  Period=4  PulseWidth=50
  Pulse Generator1 : DiscretePulseGenerator  PulseType=Time based  Amplitude=2  Period=4  PulseWidth=50
  ROLLING RESISTANCE MAGNITUDE (W FRAME) : Subsystem
      settings: PortSchema="{\"entries\":[{\"content\":{\"sides\":[{\"content\":{\"connectorIds\":[\"In1\",\"In2\"]},\"type\":\"ConnectorPlacement.EquallySpacedRectSide\",\"uuid\":\"12660b93-1e91-4304-a59f-3eeefd87b2e0\"},{\"content\":{\"connectorIds\":[\"Out1\"],\"side\":\"RIGHT\"},\"type\":\"ConnectorPlacement.EquallySpacedRectSide\",\"uuid\":\"8e6f71a0-242d-4b35-81c2-70bf2b11da18\"},{\"content\":{\"connectorIds\":[\"In3\"],\"side\":\"TOP\"},\"type\":\"ConnectorPlacement.EquallySpacedRectSide\",\"uuid\":\"1cd46535-1ca8-4592-bf34-1ae182597033\"}]},\"type\":\"ConnectorPlacement.EquallySpacedConnector\",\"uuid\":\"cae9c1b4-8a83-44d8-ab36-6e338131f762\"}],\"packageUris\":[\"http://schema.mathworks.com/mf0/Connector/R2020b\"],\"version\":\"1.0\"}"
  Radians to Degrees : simulink_extras/Transformations/Radians to Degrees
  Rolling Resistance W --> B Transformation : Subsystem
  Scope{1..4} (4 alike) : Scope
  Slip Angle and Corner Velocity : Subsystem
  Steering Kinematics : Subsystem
  Subsystem : Subsystem
  Subsystem1 : Subsystem
  Switch : Switch  Criteria=u2 > Threshold  SaturateOnIntegerOverflow=off  InputSameDT=off
  Terminator : Terminator
  Terminator1 : Terminator
  Tire Forces W --> B Transformation : Subsystem
  Tire Model Pacejka 5.2 : Subsystem
  Tire Vertical Load : Subsystem
  To Workspace : ToWorkspace  VariableName=wheelLinearSpeed  SaveFormat=Timeseries  SampleTime=-1
  To Workspace1 : ToWorkspace  VariableName=iFrame  SaveFormat=Timeseries  SampleTime=-1
  Transport Delay2 : TransportDelay  DelayTime=2  BufferSize=5120
  Velocity B --> Velocity I Transformation : Subsystem
  Wheel Dynamics : Subsystem
      settings: PortSchema="{\"entries\":[{\"content\":{\"sides\":[{\"content\":{\"connectorIds\":[\"In1\",\"In2\",\"In3\",\"In4\",\"In5\",\"In6\",\"In7\"]},\"type\":\"ConnectorPlacement.EquallySpacedRectSide\",\"uuid\":\"422fe093-17a9-4a73-963b-03d68c58349a\"},{\"content\":{\"connectorIds\":[\"Out1\",\"Out2\",\"Out3\"],\"side\":\"RIGHT\"},\"type\":\"ConnectorPlacement.EquallySpacedRectSide\",\"uuid\":\"569da465-14b9-4946-a082-557794cd3ed0\"},{\"content\":{\"connectorIds\":[\"In8\",\"In9\"],\"side\":\"TOP\"},\"type\":\"ConnectorPlacement.EquallySpacedRectSide\",\"uuid\":\"1c5b2222-0506-4f34-b7d5-3aec22bb1293\"},{\"content\":{\"connectorIds\":[\"In10\"],\"side\":\"BOTTOM\"},\"type\":\"ConnectorPlacement.EquallySpacedRectSide\",\"uuid\":\"71b45c36-892e-4acc-b3c3-cb0225fd1ae8\"}]},\"type\":\"ConnectorPlacement.EquallySpacedConnector\",\"uuid\":\"8ed83d55-5df2-44df-928e-367e127158cc\"}],\"packageUris\":[\"http://schema.mathworks.com/mf0/Connector/R2020b\"],\"version\":\"1.0\"}"
  Distance Traveled : Outport
  Speed : Outport  Port=2
  Ax_B : Outport  Port=3
  Ay_B : Outport  Port=4
  Ax_I : Outport  Port=5
  Ay_I : Outport  Port=6
  X POS_I : Outport  Port=7
  Y POS_I : Outport  Port=8
  YAW ANGLE (DEG) : Outport  Port=9
  wires:
  Slip Angle and Corner Velocity/1(Alpha) -> ALPHA (DEG)/1, [Alpha]
  Constant5/1 -> Bus Creator1/1, Bus Creator1/2, Bus Creator1/4, Bus Creator1/3
  Tire Forces W --> B Transformation/1(TIRE FORCES VECTOR (B FRAME)) -> Equations of Motion/1(TIRE FORCES VECTOR (B FRAME))
  Product/1 -> To Workspace/1  "Wheel Linear Speed"
  Divide/1 -> Terminator/1  "Ax_B (Gs)"
  [Delta_Right_Rad] -> Tire Forces W --> B Transformation/3(Delta Right), Rolling Resistance W --> B Transformation/3(Delta Right)
  Steering Kinematics/2(Delta Right) -> [Delta_Right_Rad], Wheel Dynamics/9(Delta_Right)  "Delta_Right"
  [Delta_Left_Rad] -> Longitudinal Corner Vel B --> W Transformation/1(Delta Left Rad)
  [Ay_I] -> Memory1/1
  Velocity B --> Velocity I Transformation/2(dYdt_Inertial) -> Bus Creator/4, Inertial Position Integration/2(dYdt_Inertial)  "Y VEL INERTIAL"
  Constant1/1 -> Product/2
  Tire Vertical Load/1(Fz) -> Tire Model Pacejka 5.2/3(Fz), ROLLING RESISTANCE MAGNITUDE (W FRAME)/1(Fz)
  Bus Creator/1 -> To Workspace1/1
  [Delta_Right_Rad] -> Longitudinal Corner Vel B --> W Transformation/2(Delta Right Rad)
  [Alpha] -> Tire Model Pacejka 5.2/2(Alpha), Wheel Dynamics/10(Alpha)
  [Vx_B] -> Velocity B --> Velocity I Transformation/1(dXdt_B)
  Inertial Position Integration/3(YAW ANGLE (DEG)) -> YAW ANGLE (DEG)/1, Bus Creator/5  "YAW ANGLE DEG"
  Equations of Motion/2(Vx_B) -> Subsystem1/3(Vx_B), [Vx_B]  "Vx_B"
  [Long_Corner_Vel_W] -> Wheel Dynamics/7(Longitudinal Corner Vel (W Frame)), Longitudinal Slip/3(Longitudinal Corner Vel (W Frame))
  Inertial Position Integration/1(X POS_I) -> X POS_I/1, Bus Creator/1  "X POS INERTIAL"
  Equations of Motion/3(Ay_B) -> Divide1/1, Subsystem1/2(Ay_B), Ay_B/1, [Ay_B]  "Ay_B"
  Steering Kinematics/1(Delta Left) -> [Delta_Left_Rad], Wheel Dynamics/8(Delta_Left)  "Delta_Left"
  Inertial Position Integration/2(Y POS_I) -> Y POS_I/1, Bus Creator/3  "Y POS INERTIAL"
  Radians to Degrees/1 -> Scope3/1  "Beta (DEG)"
  Equations of Motion/8(Ax_I) -> Ax_I/1, [Ax_I]  "Ax_I"
  ROLLING RESISTANCE MAGNITUDE (W FRAME)/1(ROLLING RESISTANCE (W FRAME)) -> Rolling Resistance W --> B Transformation/1(ROLLING RESISTANCE MAGNITUDE (W FRAME)), Wheel Dynamics/6(ROLLING RESISTANCE (W FRAME))
  ALPHA (DEG)/1 -> Scope4/1
  Wheel Dynamics/1(Wheel Omega) -> Product/1, ROLLING RESISTANCE MAGNITUDE (W FRAME)/2(Wheel Omega), Longitudinal Slip/1(Wheel Omega)
  Atan/1 -> Radians to Degrees/1, Velocity B --> Velocity I Transformation/4(Body Slip (RAD))
  Divide2/1 -> Atan/1
  [Delta_Left_Rad] -> Slip Angle and Corner Velocity/4(Delta Left)
  [Yaw_Rate] -> Slip Angle and Corner Velocity/3(Yaw Rate)
  Velocity B --> Velocity I Transformation/3(YAW ANGLE) -> Inertial Position Integration/3(YAW ANGLE (RAD))  "Yaw Angle (Rad)"
  Constant4/1 -> Divide/2
  [Yaw_Accel] -> Scope1/1
  Velocity B --> Velocity I Transformation/1(dXdt_Inertial) -> Bus Creator/2, Inertial Position Integration/1(dXdt_Inertial)  "X VEL INERTIAL"
  Memory/1 -> Tire Vertical Load/2(Ax_I)
  Wheel Dynamics/2(Requested Motor Torque) -> Longitudinal Slip/2(Requested Motor Torque)
  Equations of Motion/9(Ay_I) -> Ay_I/1, [Ay_I]  "Ay_I"
  [Vy_B] -> Velocity B --> Velocity I Transformation/2(dYdt_B)
  Tire Model Pacejka 5.2/1(TIRE FORCES VECTOR (W FRAME)) -> Wheel Dynamics/5(TIRE FORCES (W FRAME)), Tire Forces W --> B Transformation/1(TIRE FORCES (W FRAME))
  Memory1/1 -> Tire Vertical Load/3(Ay_I)
  [Yaw_Rate] -> Velocity B --> Velocity I Transformation/3(dYawdt)
  Constant6/1 -> Divide1/2
  [Ax_I] -> Memory/1
  Longitudinal Corner Vel B --> W Transformation/1(LONGITUDINAL CORNER VEL (W FRAME)) -> [Long_Corner_Vel_W]
  Rolling Resistance W --> B Transformation/1(ROLLING RESISTANCE VECTOR (B FRAME)) -> Equations of Motion/3(ROLLING RESISTANCE VECTOR (B FRAME))
  Tire Model Pacejka 5.2/2(TIRE MOMENT VECTOR) -> Equations of Motion/2(TIRE MOMENT VECTOR)
  Wheel Dynamics/3(Constrained Motor Torque) -> Scope2/1
  Equations of Motion/7(Speed) -> Integrator/1(Speed), [Speed], Subsystem1/7(Speed), Speed/1  "Speed"
  [Delta_Right_Rad] -> Slip Angle and Corner Velocity/5(Delta Right)
  Subsystem/1(DRAG FORCE MAGNITUDE) -> Equations of Motion/4(DRAG FORCE MAGNITUDE (B FRAME))
  [Delta_Left_Rad] -> Tire Forces W --> B Transformation/2(Delta Left), Rolling Resistance W --> B Transformation/2(Delta Left)
  Equations of Motion/6(Yaw Rate) -> Subsystem1/6(Yaw_Rate), [Yaw_Rate]  "Yaw_Rate"
  Slip Angle and Corner Velocity/2(LONGITUDINAL CORNER VEL (DIRECTION OF BODY)) -> Longitudinal Corner Vel B --> W Transformation/3(LONGITUDINAL CORNER VEL (DIRECTION OF BODY))
  Equations of Motion/4(Vy_B) -> Subsystem1/4(Vy_B), [Vy_B]  "Vy_B"
  Longitudinal Slip/1(SL) -> Tire Model Pacejka 5.2/1(SL), ROLLING RESISTANCE MAGNITUDE (W FRAME)/3(SL)
  Bus Creator1/1 -> Tire Model Pacejka 5.2/4(IA)
  Equations of Motion/1(Ax_B) -> Divide/1, Subsystem1/1(Ax_B), Ax_B/1, [Ax_B]  "Ax_B"
  [Speed] -> Tire Vertical Load/1(Speed), Subsystem/1(Speed)
  [Vx_B] -> Switch/2, Switch/1, Slip Angle and Corner Velocity/1(Vx_B)
  Equations of Motion/5(Yaw Accel.) -> Subsystem1/5(Yaw_Accel), [Yaw_Accel]  "Yaw_Accel"
  [Vy_B] -> Divide2/1, Slip Angle and Corner Velocity/2(Vy_B)
  Divide1/1 -> Terminator1/1  "Ay_B (Gs)"
  Wheel Steer Input [deg]/1 -> Memory2/1
  Integrator/1(Distance Along Track) -> Distance Traveled/1
  Memory2/1 -> Steering Kinematics/1(Delta Avg (DEG))
  Pulse Generator/1 -> Add/1
  Pulse Generator1/1 -> Transport Delay2/1
  Transport Delay2/1 -> Add/2
  Constant2/1 -> Switch/3
  Switch/1 -> Divide2/2
  FL Torque/1 -> Wheel Dynamics/1(Torque FL)
  FR Torque/1 -> Wheel Dynamics/2(Torque FR)
  RL Torque/1 -> Wheel Dynamics/3(Torque RL)
  RR Torque/1 -> Wheel Dynamics/4(Torque RR)

== system FullCarLateral/Constant Input PID ==
  Vx_B : Inport
  Wheel Delta [rad] : Inport  Port=2
  Yaw Rate [rad/s] : Inport  Port=3
  Constant{,1..3} (4 alike) : Constant  Value=5
  Gain : Gain  Gain=-1
  PID Controller : slpidlib/PID Controller  Controller=PID  Form=Parallel  TimeDomain=Discrete-time  UseExternalTs=off  SampleTime=-1  IntegratorMethod=Forward Euler  FilterMethod=Forward Euler  ControllerParametersSource=internal  P=3  I=1  UseKiTs=off  D=0  N=100  UseFilter=on  TunerSelectOption=Transfer Function Based (PID Tuner App)  InitialConditionSource=internal  InitialConditionForIntegrator=0  InitialConditionForFilter=0  DifferentiatorICPrevScaledInput=0  ExternalReset=none  TrackingMode=off  Kt=1  LimitOutput=off  SatLimitsSource=internal  UpperSaturationLimit=inf  LowerSaturationLimit=-inf  LinearizeAsGain=on  AntiWindupMode=none  Kb=1  LimitIntegrator=off  UpperIntegratorSaturationLimit=inf  LowerIntegratorSaturationLimit=-inf  POutMin=[]  POutMax=[]  IOutMin=[]  IOutMax=[]  DOutMin=[]  DOutMax=[]  NOutMin=[]  NOutMax=[]  SumOutMin=[]  SumOutMax=[]  SaturationOutMin=[]  SaturationOutMax=[]  PParamMin=[]  PParamMax=[]  IParamMin=[]  IParamMax=[]  DParamMin=[]  DParamMax=[]  NParamMin=[]  NParamMax=[]  KbParamMin=[]  KbParamMax=[]  KtParamMin=[]  KtParamMax=[]  KbOutMin=[]  KbOutMax=[]  KtOutMin=[]  KtOutMax=[]  IntegratorOutMin=[]  IntegratorOutMax=[]  FilterOutMin=[]  FilterOutMax=[]  SumI1OutMin=[]  SumI1OutMax=[]  SumI2OutMin=[]  SumI2OutMax=[]  SumI3OutMin=[]  SumI3OutMax=[]  SumI4OutMin=[]  SumI4OutMax=[]  SumDOutMin=[]  SumDOutMax=[]  DifferentiatorOutMin=[]  DifferentiatorOutMax=[]  FilterDiffOutCoefMin=[]  FilterDiffOutCoefMax=[]  ReciprocalOutMin=[]  ReciprocalOutMax=[]  SumDenOutMin=[]  SumDenOutMax=[]  SumNumOutMin=[]  SumNumOutMax=[]  DivideOutMin=[]  DivideOutMax=[]  UdiffTsProdOutMin=[]  UdiffTsProdOutMax=[]  NTsProdOutMin=[]  NTsProdOutMax=[]  UintegralTsProdOutMin=[]  UintegralTsProdOutMax=[]  UngainTsProdOutMin=[]  UngainTsProdOutMax=[]  ClampingZeroOutDataTypeStr=Inherit: Inherit via back propagation  ClampingZeroOutMin=[]  ClampingZeroOutMax=[]  FilterDenConstantOutDataTypeStr=Inherit: Inherit via back propagation  FilterDenConstantOutMin=[]  FilterDenConstantOutMax=[]  PCopyOutDataTypeStr=Inherit: Inherit via back propagation  PCopyOutMin=[]  PCopyOutMax=[]  NCopyOutDataTypeStr=Inherit: Inherit via back propagation  NCopyOutMin=[]  NCopyOutMax=[]  IntegratorContinuousStateAttributes=''  IntegratorStateMustResolveToSignalObject=off  IntegratorRTWStateStorageClass=Auto  FilterContinuousStateAttributes=''  FilterStateMustResolveToSignalObject=off  FilterRTWStateStorageClass=Auto  ParallelPVariant=InternalParameters  IdealPVariant=Disabled  IVariant=InternalParameters  DVariant=InternalParameters  IntegratorVariant=Discrete  SatVariant=Disabled  AWVariant=Passthrough  PCopyVariant=Disabled  TRVariant=Disabled  FdbkBlocksVariant=Forward  IdealPFdbkVariant=Disabled  SatFdbkVariant=Disabled  DerivativeFilterVariant=ForwardEulerFilter  NVariant=InternalParameters  NCopyVariant=Disabled  FilterICVariant=InternalICsFilter  IntegratorICVariant=InternalICs  ExternalResetVariant=Disabled  TRSumVariant=Passthrough  SumFdbkVariant=Disabled  SumVariant=Sum_PID  TsampFilterVariant=InternalTs  TsampNgainVariant=Passthrough  TsampIntegralVariant=Disabled_SignalSpec  ExternalSaturationOutDataTypeStr=Inherit: Same as second input
  Subsystem3 : Subsystem
  Sum : Sum  Inputs=|++
  Sum1 : Sum  Inputs=|++
  Sum2 : Sum  Inputs=|-+
  Sum3 : Sum  Inputs=|-+
  FR Torque After : Outport
  RR Torque After : Outport  Port=2
  FL Torque After : Outport  Port=3
  RL Torque After : Outport  Port=4
  wires:
  Sum2/1 -> FL Torque After/1  "FL Torque After"
  Sum3/1 -> RL Torque After/1  "RL Torque After"
  Constant2/1 -> Sum2/2  "FL Torque Before"
  Sum/1 -> FR Torque After/1  "FR Torque After"
  Sum1/1 -> RR Torque After/1  "RR Torque After"
  Constant3/1 -> Sum3/2  "RL Torque Before"
  Subsystem3/1(Yaw Error [rad/s]) -> PID Controller/1  "Yaw Error [rad/s]"
  Constant/1 -> Sum/2  "FR Torque Before"
  Gain/1 -> Sum/1, Sum1/1, Sum2/1, Sum3/1
  Constant1/1 -> Sum1/2  "RR Torque Before"
  PID Controller/1 -> Gain/1
  Vx_B/1 -> Subsystem3/1(Vx_B [m/s])
  Wheel Delta [rad]/1 -> Subsystem3/2(Delta [rad])
  Yaw Rate [rad/s]/1 -> Subsystem3/3(Yaw Rate [Rad/s])

== system FullCarLateral/Data Input PID ==
  From Workspace : FromWorkspace  VariableName=[timelsim motorTorqueFLInterp]
  From Workspace2 : FromWorkspace  VariableName=[timelsim motorTorqueRLInterp]
  From Workspace3 : FromWorkspace  VariableName=[timelsim motorTorqueRRInterp]
  From Workspace5 : FromWorkspace  VariableName=[timelsim motorTorqueFRInterp]
  Gain : Gain  Gain=-1
  PID Controller : slpidlib/PID Controller  Controller=PID  Form=Parallel  TimeDomain=Continuous-time  UseExternalTs=off  SampleTime=-1  IntegratorMethod=Forward Euler  FilterMethod=Forward Euler  ControllerParametersSource=internal  P=0  I=0  UseKiTs=off  D=0  N=100  UseFilter=on  TunerSelectOption=Transfer Function Based (PID Tuner App)  InitialConditionSource=internal  InitialConditionForIntegrator=0  InitialConditionForFilter=0  DifferentiatorICPrevScaledInput=0  ExternalReset=none  TrackingMode=off  Kt=1  LimitOutput=off  SatLimitsSource=internal  UpperSaturationLimit=inf  LowerSaturationLimit=-inf  LinearizeAsGain=on  AntiWindupMode=none  Kb=1  LimitIntegrator=off  UpperIntegratorSaturationLimit=inf  LowerIntegratorSaturationLimit=-inf  POutMin=[]  POutMax=[]  IOutMin=[]  IOutMax=[]  DOutMin=[]  DOutMax=[]  NOutMin=[]  NOutMax=[]  SumOutMin=[]  SumOutMax=[]  SaturationOutMin=[]  SaturationOutMax=[]  PParamMin=[]  PParamMax=[]  IParamMin=[]  IParamMax=[]  DParamMin=[]  DParamMax=[]  NParamMin=[]  NParamMax=[]  KbParamMin=[]  KbParamMax=[]  KtParamMin=[]  KtParamMax=[]  KbOutMin=[]  KbOutMax=[]  KtOutMin=[]  KtOutMax=[]  IntegratorOutMin=[]  IntegratorOutMax=[]  FilterOutMin=[]  FilterOutMax=[]  SumI1OutMin=[]  SumI1OutMax=[]  SumI2OutMin=[]  SumI2OutMax=[]  SumI3OutMin=[]  SumI3OutMax=[]  SumI4OutMin=[]  SumI4OutMax=[]  SumDOutMin=[]  SumDOutMax=[]  DifferentiatorOutMin=[]  DifferentiatorOutMax=[]  FilterDiffOutCoefMin=[]  FilterDiffOutCoefMax=[]  ReciprocalOutMin=[]  ReciprocalOutMax=[]  SumDenOutMin=[]  SumDenOutMax=[]  SumNumOutMin=[]  SumNumOutMax=[]  DivideOutMin=[]  DivideOutMax=[]  UdiffTsProdOutMin=[]  UdiffTsProdOutMax=[]  NTsProdOutMin=[]  NTsProdOutMax=[]  UintegralTsProdOutMin=[]  UintegralTsProdOutMax=[]  UngainTsProdOutMin=[]  UngainTsProdOutMax=[]  ClampingZeroOutDataTypeStr=Inherit: Inherit via back propagation  ClampingZeroOutMin=[]  ClampingZeroOutMax=[]  FilterDenConstantOutDataTypeStr=Inherit: Inherit via back propagation  FilterDenConstantOutMin=[]  FilterDenConstantOutMax=[]  PCopyOutDataTypeStr=Inherit: Inherit via back propagation  PCopyOutMin=[]  PCopyOutMax=[]  NCopyOutDataTypeStr=Inherit: Inherit via back propagation  NCopyOutMin=[]  NCopyOutMax=[]  IntegratorContinuousStateAttributes=''  IntegratorStateMustResolveToSignalObject=off  IntegratorRTWStateStorageClass=Auto  FilterContinuousStateAttributes=''  FilterStateMustResolveToSignalObject=off  FilterRTWStateStorageClass=Auto  ParallelPVariant=InternalParameters  IdealPVariant=Disabled  IVariant=InternalParameters  DVariant=InternalParameters  IntegratorVariant=Continuous  SatVariant=Disabled  AWVariant=Passthrough  PCopyVariant=Disabled  TRVariant=Disabled  FdbkBlocksVariant=Forward  IdealPFdbkVariant=Disabled  SatFdbkVariant=Disabled  DerivativeFilterVariant=ContFilter  NVariant=InternalParameters  NCopyVariant=Disabled  FilterICVariant=InternalICsFilter  IntegratorICVariant=InternalICs  ExternalResetVariant=Disabled  TRSumVariant=Passthrough  SumFdbkVariant=Disabled  SumVariant=Sum_PID  TsampFilterVariant=InternalTs  TsampNgainVariant=Passthrough  TsampIntegralVariant=Disabled_SignalSpec  ExternalSaturationOutDataTypeStr=Inherit: Same as second input
  Subsystem3 : Subsystem
  Sum : Sum  Inputs=|++
  Sum1 : Sum  Inputs=|++
  Sum2 : Sum  Inputs=|-+
  Sum3 : Sum  Inputs=|-+
  FR Torque After : Outport
  RR Torque After : Outport  Port=2
  FL Torque After : Outport  Port=3
  RL Torque After : Outport  Port=4
  wires:
  PID Controller/1 -> Gain/1
  [Delta_Left_Rad] -> Subsystem3/2(Delta [rad])
  [Yaw_Rate] -> Subsystem3/3(Yaw Rate [Rad/s])
  From Workspace3/1 -> Sum1/2  "RR Torque Before"
  Gain/1 -> Sum3/1, Sum2/1, Sum1/1, Sum/1
  From Workspace5/1 -> Sum/2  "FR Torque Before"
  Subsystem3/1(Yaw Error [rad/s]) -> PID Controller/1  "Yaw Error [rad/s]"
  From Workspace2/1 -> Sum3/2  "RL Torque Before"
  Sum1/1 -> RR Torque After/1  "RR Torque After"
  [Vx_B] -> Subsystem3/1(Vx_B [m/s])
  Sum/1 -> FR Torque After/1  "FR Torque After"
  From Workspace/1 -> Sum2/2  "FL Torque Before"
  Sum3/1 -> RL Torque After/1  "RL Torque After"
  Sum2/1 -> FL Torque After/1  "FL Torque After"

== system FullCarLateral/Stop Simulation Based on Distance ==
  Distance Traveled : Inport
  Constant2 : Constant  Value=trackReference.length
  Constant3 : Constant
  Constant4 : Constant  Value=0
  If : If  NumInputs=2  IfExpression=u1 >= u2
  If Action Subsystem : Subsystem  TreatAsAtomicUnit=on
  If Action Subsystem1 : Subsystem  TreatAsAtomicUnit=on
  Merge : Merge
  Stop Simulation : Stop
  wires:
  Constant4/1 -> If Action Subsystem1/1(In1)
  Merge/1 -> Stop Simulation/1
  If Action Subsystem/1(Out1) -> Merge/1
  Constant2/1 -> If/2
  If/1 -> If Action Subsystem/Action
  If/2 -> If Action Subsystem1/Action
  If Action Subsystem1/1(Out1) -> Merge/2
  Constant3/1 -> If Action Subsystem/1(In1)
  Distance Traveled/1 -> If/1

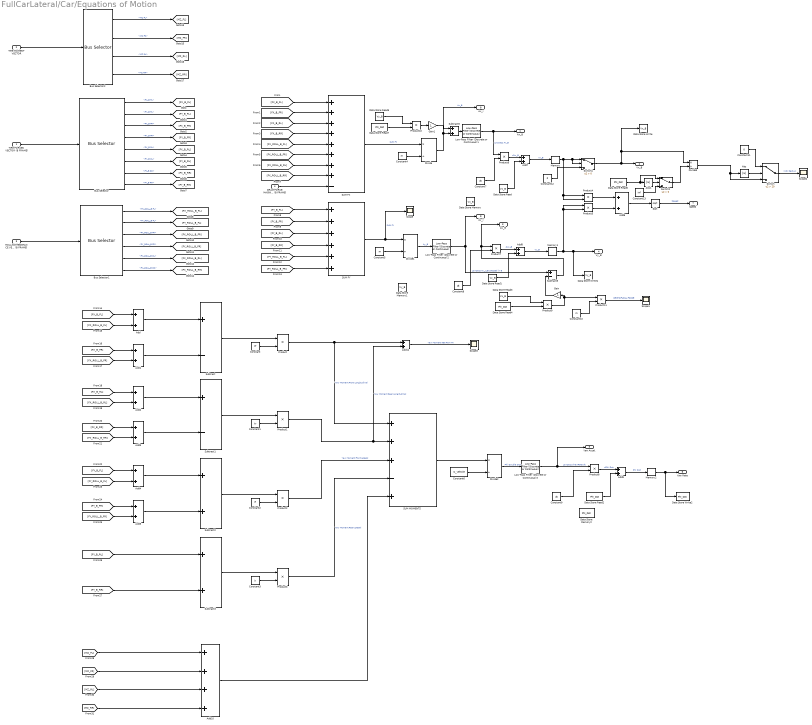
== system FullCarLateral/Car/Equations of Motion ==
  TIRE FORCES VECTOR (B FRAME) : Inport
  TIRE MOMENT VECTOR : Inport  Port=2
  ROLLING RESISTANCE VECTOR (B FRAME) : Inport  Port=3
  DRAG FORCE MAGNITUDE (B FRAME) : Inport  Port=4
  Abs : Abs  SaturateOnIntegerOverflow=off
  Abs1 : Abs  SaturateOnIntegerOverflow=off
  Add{,1..9,11} (11 alike) : Sum
  Add10 : Sum  Inputs=++++
  Bus Selector : BusSelector  OutputSignals=FX_B FL,FY_B FL,FX_B FR,FY_B FR,FX_B RL,FY_B RL,FX_B RR,FY_B RR
  Bus Selector1 : BusSelector  OutputSignals=FX_ROLL_B FL,FY_ROLL_B FL,FX_ROLL_B FR,FY_ROLL_B FR,FX_ROLL_B RL,FX_ROLL_B RR
  Bus Selector2 : BusSelector  OutputSignals=MZ FL,MZ FR,MZ RL,MZ RR
  Constant : Constant  Value=tf
  Constant1 : Constant  Value=tr
  Constant10 : Constant  Value=m
  Constant11 : Constant  Value=0
  Constant12 : Constant  Value=0
  Constant13 : Constant  Value=inf
  Constant2 : Constant  Value=lf
  Constant3 : Constant  Value=lr
  Constant4 : Constant  Value=m
  Constant5 : Constant  Value=m
  Constant6 : Constant  Value=Iz_vehicle
  Constant7 : Constant  Value=dt
  Constant8 : Constant  Value=dt
  Constant9 : Constant  Value=dt
  Data Store Memory : DataStoreMemory  DataStoreName=Vx_B  WriteAfterWriteMsg=warning  ShowAdditionalParam=off
  Data Store Memory1 : DataStoreMemory  DataStoreName=Vy_B  WriteAfterWriteMsg=warning  ShowAdditionalParam=off
  Data Store Memory2 : DataStoreMemory  DataStoreName=Phi_Dot  WriteAfterWriteMsg=warning  ShowAdditionalParam=off
  Data Store Read : DataStoreRead  DataStoreName=Vx_B  IndexOptions=Index vector (dialog)  Indices=1  OutputSizes=1
  Data Store Read1 : DataStoreRead  DataStoreName=Vy_B  IndexOptions=Index vector (dialog)  Indices=1  OutputSizes=1
  Data Store Read{2,4,6..7} (4 alike) : DataStoreRead  DataStoreName=Phi_Dot  IndexOptions=Index vector (dialog)  Indices=1  OutputSizes=1
  Data Store Read3 : DataStoreRead  DataStoreName=Vx_B  IndexOptions=Index vector (dialog)  Indices=1  OutputSizes=1
  Data Store Read5 : DataStoreRead  DataStoreName=Vy_B  IndexOptions=Index vector (dialog)  Indices=1  OutputSizes=1
  Data Store Write : DataStoreWrite  DataStoreName=Vx_B  IndexOptions=Index vector (dialog)  Indices=1  OutputSizes=1
  Data Store Write1 : DataStoreWrite  DataStoreName=Vy_B  IndexOptions=Index vector (dialog)  Indices=1  OutputSizes=1
  Data Store Write2 : DataStoreWrite  DataStoreName=Phi_Dot  IndexOptions=Index vector (dialog)  Indices=1  OutputSizes=1
  Divide{,1..3} (4 alike) : Product  Inputs=*/
  Gain : Gain
  Gain1 : Gain
  Low-Pass Filter (Discrete or Continuous)1 : eeGeneralControl/Low-Pass Filter (Discrete or Continuous)  K=1  T=lowpassT  B=inf  A=-inf  init_option=Inherited from block input  x0=0  Ts=-1
  Low-Pass Filter (Discrete or Continuous)2 : eeGeneralControl/Low-Pass Filter (Discrete or Continuous)  K=1  T=lowpassT  B=inf  A=-inf  init_option=Inherited from block input  x0=0  Ts=-1
  Low-Pass Filter (Discrete or Continuous)3 : eeGeneralControl/Low-Pass Filter (Discrete or Continuous)  K=1  T=lowpassT  B=inf  A=-inf  init_option=Inherited from block input  x0=0  Ts=-1
  Memory : Memory
  Memory1 : Memory
  Memory2 : Memory
  Product{,1..11} (12 alike) : Product
  SUM FX : Sum  Inputs=++++++++-
  SUM FY : Sum  Inputs=++++++
  SUM MOMENTS : Sum  Inputs=+++-+
  Scope{,1..3} (4 alike) : Scope
  Sqrt : Sqrt
  Subtract : Sum  Inputs=+-
  Subtract1 : Sum  Inputs=+-
  Subtract2 : Sum
  Subtract3 : Sum
  Subtract5 : Sum  Inputs=+-
  Subtract6 : Sum
  Switch : Switch  Criteria=u2 > Threshold  Threshold=20  SaturateOnIntegerOverflow=off  InputSameDT=off
  Switch1 : Switch  Criteria=u2 > Threshold  SaturateOnIntegerOverflow=off  InputSameDT=off
  Switch2 : Switch  Criteria=u2 > Threshold  SaturateOnIntegerOverflow=off  InputSameDT=off
  Ax_B : Outport
  Vx_B : Outport  Port=2
  Ay_B : Outport  Port=3
  Vy_B : Outport  Port=4
  Yaw Accel. : Outport  Port=5
  Yaw Rate : Outport  Port=6
  Speed : Outport  Port=7
  Ax_I : Outport  Port=8
  Ay_I : Outport  Port=9
  wires:
  TIRE FORCES VECTOR (B FRAME)/1 -> Bus Selector/1
  ROLLING RESISTANCE VECTOR (B FRAME)/1 -> Bus Selector1/1
  Bus Selector/2 -> [FY_B_FL]  "<FY_B FL>"
  Bus Selector/4 -> [FY_B_FR]  "<FY_B FR>"
  Bus Selector/6 -> [FY_B_RL]  "<FY_B RL>"
  Bus Selector/8 -> [FY_B_RR]  "<FY_B RR>"
  Bus Selector1/2 -> [FY_ROLL_B_FL]  "<FY_ROLL_B FL>"
  Bus Selector1/4 -> [FY_ROLL_B_FR]  "<FY_ROLL_B FR>"
  Bus Selector/1 -> [FX_B_FL]  "<FX_B FL>"
  Bus Selector1/1 -> [FX_ROLL_B_FL]  "<FX_ROLL_B FL>"
  Bus Selector/3 -> [FX_B_FR]  "<FX_B FR>"
  Bus Selector/5 -> [FX_B_RL]  "<FX_B RL>"
  Bus Selector/7 -> [FX_B_RR]  "<FX_B RR>"
  Bus Selector1/3 -> [FX_ROLL_B_FR]  "<FX_ROLL_B FR>"
  Bus Selector1/5 -> [FX_ROLL_B_RL]  "<FX_ROLL_B RL>"
  Bus Selector1/6 -> [FX_ROLL_B_RR]  "<FX_ROLL_B RR>"
  [FX_B_FL] -> SUM FX/1
  DRAG FORCE MAGNITUDE (B FRAME)/1 -> SUM FX/9
  [FX_B_FR] -> SUM FX/2
  [FX_B_RL] -> SUM FX/3
  [FX_B_RR] -> SUM FX/4
  [FX_ROLL_B_RL] -> SUM FX/7
  [FX_ROLL_B_RR] -> SUM FX/8
  [FY_B_FL] -> SUM FY/1
  [FY_B_FR] -> SUM FY/2
  [FY_B_RL] -> SUM FY/3
  [FY_B_RR] -> SUM FY/4
  [FY_ROLL_B_FL] -> SUM FY/5
  [FY_ROLL_B_FR] -> SUM FY/6
  SUM FX/1 -> Divide/1  "SUM FX"
  [FX_B_FL] -> Add/1
  [FX_ROLL_B_FL] -> Add/2
  [FX_ROLL_B_FR] -> Add1/2
  [FX_B_FR] -> Add1/1
  [FX_B_RL] -> Add2/1
  [FX_ROLL_B_RL] -> Add2/2
  [FX_ROLL_B_RR] -> Add3/2
  [FX_B_RR] -> Add3/1
  [FY_B_FL] -> Add4/1
  [FY_ROLL_B_FL] -> Add4/2
  [FY_ROLL_B_FR] -> Add5/2
  [FY_B_FR] -> Add5/1
  Add/1 -> Subtract/1
  Add1/1 -> Subtract/2
  Subtract/1 -> Product/1
  Constant/1 -> Product/2
  Constant1/1 -> Product1/2
  Subtract1/1 -> Product1/1
  Add2/1 -> Subtract1/1
  Add3/1 -> Subtract1/2
  Subtract2/1 -> Product2/1
  Constant2/1 -> Product2/2
  Add4/1 -> Subtract2/1
  Add5/1 -> Subtract2/2
  Constant3/1 -> Product3/2
  Subtract3/1 -> Product3/1
  [FY_B_RL] -> Subtract3/1
  [FY_B_RR] -> Subtract3/2
  Product/1 -> Add11/1, SUM MOMENTS/1  "Yaw Moment Front Longitudinal"
  Product1/1 -> Add11/2, SUM MOMENTS/2  "Yaw Moment Rear Longitudinal"
  Product2/1 -> SUM MOMENTS/3  "Yaw Moment Front Lateral"
  Product3/1 -> SUM MOMENTS/4  "Yaw Moment Rear Lateral"
  Constant4/1 -> Divide/2
  Constant5/1 -> Divide1/2
  Constant6/1 -> Divide2/2
  Divide2/1 -> Low-Pass Filter (Discrete or Continuous)3/1  "Phi Double Dot"
  Add7/1 -> Memory/1  "Vx_B"
  Add8/1 -> Memory1/1  "Vy_B"
  Add9/1 -> Memory2/1  "Phi Dot"
  Product4/1 -> Add6/1
  Product5/1 -> Add6/2
  Add6/1 -> Sqrt/1
  Sqrt/1 -> Speed/1  "Speed"
  Constant7/1 -> Product6/2
  Product6/1 -> Add7/1  "dVx_B"
  Data Store Read/1 -> Add7/2
  Constant8/1 -> Product7/2
  Product7/1 -> Add8/1  "dVy_B"
  Data Store Read1/1 -> Add8/2
  Constant9/1 -> Product8/2
  Product8/1 -> Add9/1  "dPhi Dot"
  Data Store Read2/1 -> Add9/2
  Memory/1 -> Switch1/2, Switch1/1, Product4/2, Product4/1
  Memory1/1 -> Product5/2, Product5/1, Data Store Write1/1, Vy_B/1
  [FX_ROLL_B_FL] -> SUM FX/5
  [FX_ROLL_B_FR] -> SUM FX/6
  SUM FY/1 -> Scope/1, Divide1/1  "SUM FY"
  SUM MOMENTS/1 -> Divide2/1
  Divide1/1 -> Low-Pass Filter (Discrete or Continuous)2/1  "Ay_B"
  Subtract5/1 -> Ay_B/1, Product7/1
  Divide/1 -> Subtract6/2, Ax_I/1  "Ax_B"
  Constant10/1 -> Product11/2
  Product11/1 -> Scope1/1  "CENTRIFUGAL FORCE"
  Memory2/1 -> Data Store Write2/1, Yaw Rate/1
  Product9/1 -> Product11/1, Gain/1
  Data Store Read4/1 -> Product9/2
  Data Store Read3/1 -> Product9/1
  Data Store Read5/1 -> Product10/1
  Product10/1 -> Gain1/1
  Data Store Read7/1 -> Product10/2
  Gain/1 -> Subtract5/2
  Gain1/1 -> Subtract6/1
  TIRE MOMENT VECTOR/1 -> Bus Selector2/1
  Bus Selector2/1 -> [MZ_FL]  "<MZ FL>"
  Bus Selector2/2 -> [MZ_FR]  "<MZ FR>"
  Bus Selector2/3 -> [MZ_RL]  "<MZ RL>"
  Bus Selector2/4 -> [MZ_RR]  "<MZ RR>"
  [MZ_FL] -> Add10/1
  [MZ_FR] -> Add10/2
  [MZ_RL] -> Add10/3
  [MZ_RR] -> Add10/4
  Add10/1 -> SUM MOMENTS/5
  Divide3/1 -> Abs/1, Switch/3
  Switch/1 -> Scope2/1  "Inst. Radius"
  Abs/1 -> Switch/2
  Constant11/1 -> Switch/1
  Add11/1 -> Scope3/1  "Yaw Moment Net From FX"
  Switch1/1 -> Data Store Write/1, Divide3/1, Vx_B/1
  Constant12/1 -> Switch1/3
  Data Store Read6/1 -> Switch2/1, Abs1/1
  Abs1/1 -> Switch2/2
  Switch2/1 -> Divide3/2
  Constant13/1 -> Switch2/3
  Subtract6/1 -> Low-Pass Filter (Discrete or Continuous)1/1
  Low-Pass Filter (Discrete or Continuous)1/1 -> Product6/1, Ax_B/1  "Lowpass Ax_B"
  Low-Pass Filter (Discrete or Continuous)2/1 -> Ay_I/1, Subtract5/1  "Lowpass Ay_I_Expressed in B"
  Low-Pass Filter (Discrete or Continuous)3/1 -> Product8/1, Yaw Accel./1  "Lowpass dYawRate dt"

== system FullCarLateral/Car/Inertial Position Integration ==
  dXdt_Inertial : Inport
  dYdt_Inertial : Inport  Port=2
  YAW ANGLE (RAD) : Inport  Port=3  Unit=rad
  Add1 : Sum
  Add2 : Sum
  Constant3 : Constant  Value=dt
  Constant4 : Constant  Value=dt
  Memory : Memory
  Memory1 : Memory
  Product4 : Product
  Product5 : Product
  Radians to Degrees : simulink_extras/Transformations/Radians to Degrees
  X POS_I : Outport  Unit=m
  Y POS_I : Outport  Port=2  Unit=m
  YAW ANGLE (DEG) : Outport  Port=3  Unit=deg
  wires:
  YAW ANGLE (RAD)/1 -> Radians to Degrees/1
  Radians to Degrees/1 -> YAW ANGLE (DEG)/1
  dXdt_Inertial/1 -> Product4/1
  dYdt_Inertial/1 -> Product5/1
  Add1/1 -> Memory/1
  Add2/1 -> Memory1/1
  Constant4/1 -> Product5/2
  Constant3/1 -> Product4/2
  Product5/1 -> Add2/1  "dy"
  Product4/1 -> Add1/1  "dx"
  Memory/1 -> Add1/2, X POS_I/1
  Memory1/1 -> Add2/2, Y POS_I/1

== system FullCarLateral/Car/Integrator ==
  Speed : Inport
  Add : Sum
  Constant : Constant  Value=dt
  Memory2 : Memory
  Product1 : Product
  Distance Along Track : Outport
  wires:
  Constant/1 -> Product1/2
  Memory2/1 -> Distance Along Track/1, Add/2
  Speed/1 -> Product1/1
  Product1/1 -> Add/1
  Add/1 -> Memory2/1

== system FullCarLateral/Car/Longitudinal Corner Vel B --> W Transformation ==
  Delta Left Rad : Inport
  Delta Right Rad : Inport  Port=2
  LONGITUDINAL CORNER VEL (DIRECTION OF BODY) : Inport  Port=3
  Abs : Abs  SaturateOnIntegerOverflow=off
  Abs1 : Abs  SaturateOnIntegerOverflow=off
  Bus Creator : BusCreator  Inputs=4
  Bus Selector : BusSelector  OutputSignals=LongCornerVel_FL_B,LongCornerVel_FR_B,LongCornerVel_RL_B,LongCornerVel_RR_B
  Cos : Trigonometry  Operator=cos
  Cos1 : Trigonometry  Operator=cos
  Product : Product
  Product1 : Product
  LONGITUDINAL CORNER VEL (W FRAME) : Outport
  wires:
  LONGITUDINAL CORNER VEL (DIRECTION OF BODY)/1 -> Bus Selector/1
  Bus Selector/1 -> [LongCornerVel_FL_B]  "<LongCornerVel_FL_B>"
  Bus Selector/2 -> [LongCornerVel_FR_B]  "<LongCornerVel_FR_B>"
  Bus Selector/3 -> [LongCornerVel_RL_B]  "<LongCornerVel_RL_B>"
  Bus Selector/4 -> [LongCornerVel_RR_B]  "<LongCornerVel_RR_B>"
  Delta Left Rad/1 -> Abs/1
  Delta Right Rad/1 -> Abs1/1
  Abs/1 -> Cos/1
  Abs1/1 -> Cos1/1
  Cos/1 -> [cosDeltaLeftABS]
  Cos1/1 -> [cosDeltaRightABS]
  [LongCornerVel_FL_B] -> Product/1
  [cosDeltaLeftABS] -> Product/2
  Product/1 -> Bus Creator/1  "Longitudinal_Corner_Vel_W FL"
  Product1/1 -> Bus Creator/2  "Longitudinal_Corner_Vel_W FR"
  [cosDeltaRightABS] -> Product1/2
  [LongCornerVel_FR_B] -> Product1/1
  [LongCornerVel_RL_B] -> Bus Creator/3  "Longitudinal_Corner_Vel_W RL"
  [LongCornerVel_RR_B] -> Bus Creator/4  "Longtidutinal_Corner_Vel_W RR"
  Bus Creator/1 -> LONGITUDINAL CORNER VEL (W FRAME)/1

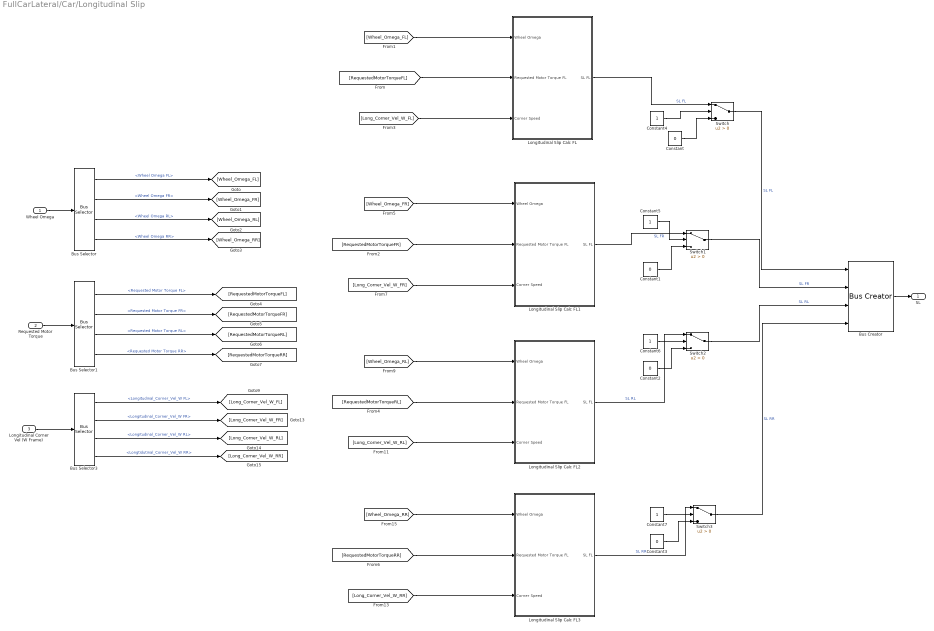
== system FullCarLateral/Car/Longitudinal Slip ==
  Wheel Omega : Inport
  Requested Motor Torque : Inport  Port=2
  Longitudinal Corner Vel (W Frame) : Inport  Port=3
  Bus Creator : BusCreator  Inputs=4
  Bus Selector : BusSelector  OutputSignals=Wheel Omega FL,Wheel Omega FR,Wheel Omega RL,Wheel Omega RR
  Bus Selector1 : BusSelector  OutputSignals=Requested Motor Torque FL,Requested Motor Torque FR,Requested Motor Torque RL,Requested Motor Torque RR
  Bus Selector3 : BusSelector  OutputSignals=Longitudinal_Corner_Vel_W FL,Longitudinal_Corner_Vel_W FR,Longitudinal_Corner_Vel_W RL,Longtidutinal_Corner_Vel_W RR
  Constant{,1..3} (4 alike) : Constant  Value=0
  Constant{4..7} (4 alike) : Constant
  Longitudinal Slip Calc FL : Subsystem
  Longitudinal Slip Calc FL1 : Subsystem
  Longitudinal Slip Calc FL2 : Subsystem
  Longitudinal Slip Calc FL3 : Subsystem
  Switch{,1..3} (4 alike) : Switch  Criteria=u2 > Threshold  SaturateOnIntegerOverflow=off  InputSameDT=off
  SL : Outport
  wires:
  Wheel Omega/1 -> Bus Selector/1
  Bus Selector/1 -> [Wheel_Omega_FL]  "<Wheel Omega FL>"
  Bus Selector/2 -> [Wheel_Omega_FR]  "<Wheel Omega FR>"
  Bus Selector/3 -> [Wheel_Omega_RL]  "<Wheel Omega RL>"
  Bus Selector/4 -> [Wheel_Omega_RR]  "<Wheel Omega RR>"
  Longitudinal Corner Vel (W Frame)/1 -> Bus Selector3/1
  [Long_Corner_Vel_W_FL] -> Longitudinal Slip Calc FL/3(Corner Speed)
  [Long_Corner_Vel_W_FR] -> Longitudinal Slip Calc FL1/3(Corner Speed)
  [Wheel_Omega_FR] -> Longitudinal Slip Calc FL1/1(Wheel Omega)
  [Wheel_Omega_RL] -> Longitudinal Slip Calc FL2/1(Wheel Omega)
  [Long_Corner_Vel_W_RL] -> Longitudinal Slip Calc FL2/3(Corner Speed)
  [Long_Corner_Vel_W_RR] -> Longitudinal Slip Calc FL3/3(Corner Speed)
  [Wheel_Omega_RR] -> Longitudinal Slip Calc FL3/1(Wheel Omega)
  Longitudinal Slip Calc FL/1(SL FL) -> Switch/1  "SL FL"
  Bus Creator/1 -> SL/1
  Bus Selector3/1 -> [Long_Corner_Vel_W_FL]  "<Longitudinal_Corner_Vel_W FL>"
  Bus Selector3/2 -> [Long_Corner_Vel_W_FR]  "<Longitudinal_Corner_Vel_W FR>"
  Bus Selector3/3 -> [Long_Corner_Vel_W_RL]  "<Longitudinal_Corner_Vel_W RL>"
  Bus Selector3/4 -> [Long_Corner_Vel_W_RR]  "<Longtidutinal_Corner_Vel_W RR>"
  [Wheel_Omega_FL] -> Longitudinal Slip Calc FL/1(Wheel Omega)
  Switch/1 -> Bus Creator/1  "SL FL"
  Constant/1 -> Switch/3
  Constant1/1 -> Switch1/3
  Constant2/1 -> Switch2/3
  Constant3/1 -> Switch3/3
  Longitudinal Slip Calc FL1/1(SL FL) -> Switch1/1  "SL FR"
  Switch1/1 -> Bus Creator/2  "SL FR"
  Switch2/1 -> Bus Creator/3  "SL RL"
  Longitudinal Slip Calc FL3/1(SL FL) -> Switch3/1  "SL RR"
  Switch3/1 -> Bus Creator/4  "SL RR"
  Requested Motor Torque/1 -> Bus Selector1/1
  Bus Selector1/1 -> [RequestedMotorTorqueFL]  "<Requested Motor Torque FL>"
  Bus Selector1/3 -> [RequestedMotorTorqueRL]  "<Requested Motor Torque RL>"
  Bus Selector1/2 -> [RequestedMotorTorqueFR]  "<Requested Motor Torque FR>"
  Bus Selector1/4 -> [RequestedMotorTorqueRR]  "<Requested Motor Torque RR>"
  [RequestedMotorTorqueFL] -> Longitudinal Slip Calc FL/2(Requested Motor Torque FL)
  [RequestedMotorTorqueFR] -> Longitudinal Slip Calc FL1/2(Requested Motor Torque FL)
  [RequestedMotorTorqueRL] -> Longitudinal Slip Calc FL2/2(Requested Motor Torque FL)
  [RequestedMotorTorqueRR] -> Longitudinal Slip Calc FL3/2(Requested Motor Torque FL)
  Constant4/1 -> Switch/2
  Constant5/1 -> Switch1/2
  Constant7/1 -> Switch3/2
  Constant6/1 -> Switch2/2
  Longitudinal Slip Calc FL2/1(SL FL) -> Switch2/1  "SL RL"

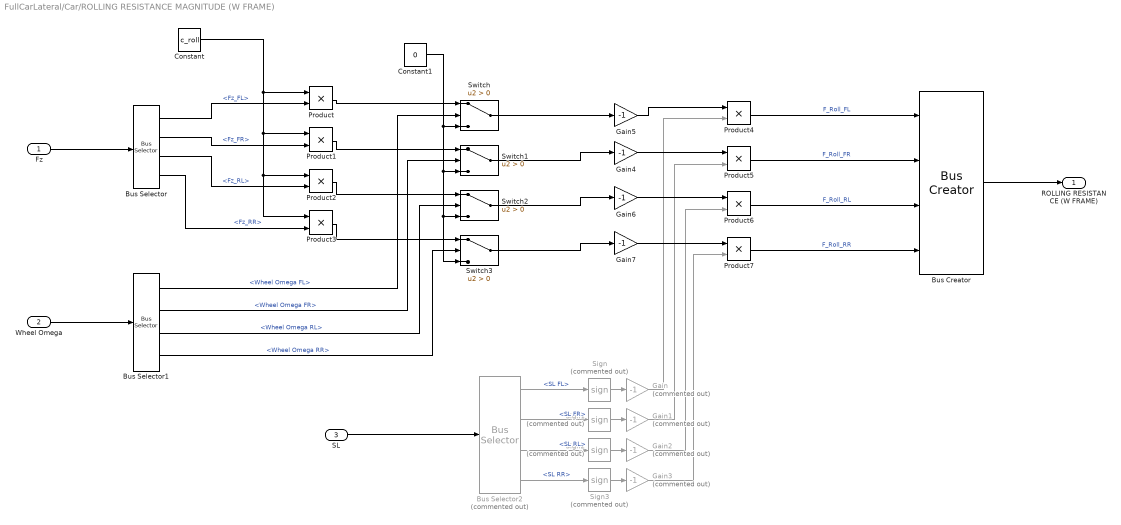
== system FullCarLateral/Car/ROLLING RESISTANCE MAGNITUDE (W FRAME) ==
  Fz : Inport
  Wheel Omega : Inport  Port=2
  SL : Inport  Port=3
  Bus Creator : BusCreator  Inputs=4
  Bus Selector : BusSelector  OutputSignals=Fz_FL,Fz_FR,Fz_RL,Fz_RR
  Bus Selector1 : BusSelector  OutputSignals=Wheel Omega FL,Wheel Omega FR,Wheel Omega RL,Wheel Omega RR
  Bus Selector2 : BusSelector  Commented=on  OutputSignals=SL FL,SL FR,SL RL,SL RR
  Constant : Constant  Value=c_roll
  Constant1 : Constant  Value=0
  Gain{,1..3} (4 alike) : Gain  Commented=on  Gain=-1
  Gain{4..7} (4 alike) : Gain  Gain=-1
  Product{,1..7} (8 alike) : Product
  Sign{,1..3} (4 alike) : Signum  Commented=on
  Switch{,1..3} (4 alike) : Switch  Criteria=u2 > Threshold  SaturateOnIntegerOverflow=off  InputSameDT=off
  ROLLING RESISTANCE (W FRAME) : Outport
  wires:
  Fz/1 -> Bus Selector/1
  Bus Selector/1 -> Product/2  "<Fz_FL>"
  Constant/1 -> Product1/1, Product2/1, Product3/1, Product/1
  Bus Creator/1 -> ROLLING RESISTANCE (W FRAME)/1
  Bus Selector/2 -> Product1/2  "<Fz_FR>"
  Bus Selector/3 -> Product2/2  "<Fz_RL>"
  Bus Selector/4 -> Product3/2  "<Fz_RR>"
  Wheel Omega/1 -> Bus Selector1/1
  Product/1 -> Switch/1
  Bus Selector1/1 -> Switch/2  "<Wheel Omega FL>"
  Constant1/1 -> Switch3/3, Switch2/3, Switch1/3, Switch/3
  Product1/1 -> Switch1/1
  Product2/1 -> Switch2/1
  Product3/1 -> Switch3/1
  Bus Selector1/2 -> Switch1/2  "<Wheel Omega FR>"
  Bus Selector1/3 -> Switch2/2  "<Wheel Omega RL>"
  Bus Selector1/4 -> Switch3/2  "<Wheel Omega RR>"
  SL/1 -> Bus Selector2/1
  Switch/1 -> Gain5/1
  Bus Selector2/1 -> Sign/1  "<SL FL>"
  Bus Selector2/2 -> Sign1/1  "<SL FR>"
  Bus Selector2/3 -> Sign2/1  "<SL RL>"
  Bus Selector2/4 -> Sign3/1  "<SL RR>"
  Sign/1 -> Gain/1
  Product4/1 -> Bus Creator/1  "F_Roll_FL"
  Product5/1 -> Bus Creator/2  "F_Roll_FR"
  Product6/1 -> Bus Creator/3  "F_Roll_RL"
  Product7/1 -> Bus Creator/4  "F_Roll_RR"
  Sign1/1 -> Gain1/1
  Sign2/1 -> Gain2/1
  Sign3/1 -> Gain3/1
  Switch1/1 -> Gain4/1
  Switch2/1 -> Gain6/1
  Switch3/1 -> Gain7/1
  Gain/1 -> Product4/2
  Gain1/1 -> Product5/2
  Gain2/1 -> Product6/2
  Gain3/1 -> Product7/2
  Gain5/1 -> Product4/1
  Gain4/1 -> Product5/1
  Gain6/1 -> Product6/1
  Gain7/1 -> Product7/1
